simulink model "sim_tase_2025_pos_ctrl"  (R2020a)
settings: Solver=ode4  StartTime=0.0  StopTime=30.0  FixedStep=0.01  RelTol=1e-3
values from neighbouring files (symbols this model uses):
  alfa_theta_obs = 100    [init_tase_2025_pos_ctrl.m]
  Aps = -diag([5, 5, 5])    [init_tase_2025_pos_ctrl.m]
  delta_p_i_0 = zeros(3, NF)    [init_tase_2025_pos_ctrl.m]
  delta_v_i_0 = zeros(3, NF)    [init_tase_2025_pos_ctrl.m]
  dp_aa_t = 0.2 * ones(3, 5) + ( 1.0 - 0.2 ) * rand(3, 5)    [init_tase_2025_pos_ctrl.m]
  dp_ff_t = [ 0.4 * ones(1, 5) + ( 1.0 - 0.4 ) * rand(1, 5);                      0.4 * ones(1, 5) + ( 1.0 - 0.4 ) * rand(1, 5);                      0.2 * ones(1, 5) + ( 0.6 - 0.2 ) * rand(1, 5) ]    [init_tase_2025_pos_ctrl.m]
  dp_phi_t = ( - pi / 2 ) * ones(3, 5) + ( pi / 2 - ( - pi / 2 ) ) * rand(3, 5)    [init_tase_2025_pos_ctrl.m]
  etai_0 = zeros(3,5)    [init_tase_2025_pos_ctrl.m]
  k_rho_1 = 10    [init_tase_2025_pos_ctrl.m]
  k_rho_2 = 10    [init_tase_2025_pos_ctrl.m]
  kai_1_t = 0.02    [init_tase_2025_pos_ctrl.m]
  kai_3_t = 0.1    [init_tase_2025_pos_ctrl.m]
  kp = 20    [init_tase_2025_pos_ctrl.m]
  ksii_0 = zeros(3,5)    [init_tase_2025_pos_ctrl.m]
  kv = 20    [init_tase_2025_pos_ctrl.m]
  l1v = diag([20; 20; 20])    [init_tase_2025_pos_ctrl.m]
  l2v = diag([30; 30; 30])    [init_tase_2025_pos_ctrl.m]
  mass_i = zeros(1,NF)    [init_tase_2025_pos_ctrl.m]
  Mii = diag([1;0;0;0;1])    [init_tase_2025_pos_ctrl.m]
  Phi_inv = inv( Aps ) * ( exp( Aps * tTs ) - eye(3) )    [init_tase_2025_pos_ctrl.m]
  pos0 = zeros(3, 1)    [init_tase_2025_pos_ctrl.m]
  PZ0 = P0(3)    [init_tase_2025_pos_ctrl.m]
  PZ1 = 10    [init_tase_2025_pos_ctrl.m]
  Qci_init = repmat([1;0;0;0],1,NF)    [init_tase_2025_pos_ctrl.m]
  R0 = 4    [init_tase_2025_pos_ctrl.m]
  R1 = 8    [init_tase_2025_pos_ctrl.m]
  Rx2 = 10    [init_tase_2025_pos_ctrl.m]
  Ry2 = 6    [init_tase_2025_pos_ctrl.m]
  Rz2 = 4    [init_tase_2025_pos_ctrl.m]
  T0 = 0    [init_tase_2025_pos_ctrl.m]
  T1 = tseq1    (= 10)    [init_tase_2025_pos_ctrl.m]
  T12 = tseq1 + tseq12    (= 20)    [init_tase_2025_pos_ctrl.m]
  T2 = tseq1 + tseq12 + tseq2    (= 30)    [init_tase_2025_pos_ctrl.m]
  theta0 = ( 2 / 5 ) * pi    (= 1.25663706144)    [init_tase_2025_pos_ctrl.m]
  theta_1 = 0    [init_tase_2025_pos_ctrl.m]
  theta_2 = 1    [init_tase_2025_pos_ctrl.m]
  TTb = 2    [init_tase_2025_pos_ctrl.m]
  tTs = 0.1    [init_tase_2025_pos_ctrl.m]
  vel0 = zeros(3, 1)    [init_tase_2025_pos_ctrl.m]
  Wij = [0,0,1,0,0;              0,0,1,1,0;              1,0,0,0,1;              0,1,1,0,0;              0,0,1,0,0]    [init_tase_2025_pos_ctrl.m]
  wp = 10    [init_tase_2025_pos_ctrl.m]
  X1 = 8    [init_tase_2025_pos_ctrl.m]
  X2 = 2    [init_tase_2025_pos_ctrl.m]
  X3 = 3    [init_tase_2025_pos_ctrl.m]
  Y1 = 10    [init_tase_2025_pos_ctrl.m]
  Y2 = 2    [init_tase_2025_pos_ctrl.m]
  Y3 = 4    [init_tase_2025_pos_ctrl.m]
  Z1 = 4    [init_tase_2025_pos_ctrl.m]
  Z2 = -6    [init_tase_2025_pos_ctrl.m]
  Z3 = 2    [init_tase_2025_pos_ctrl.m]
undefined symbols (not defined in the file or in its folder): cal_frac_squ, p_gamma1_pos, p_gamma1_vel, p_gamma2_pos, p_gamma2_vel, p_gamma_diff_1, p_gamma_diff_2_2, q_gamma1_pos, q_gamma1_vel, q_gamma2_pos, q_gamma2_vel, q_gamma_diff_1, q_gamma_diff_2_2
(part 1 of 4)
settings Model: Creator=zzy  LastModifiedBy=Hershey.A
settings DataIOCC: ReturnWorkspaceOutputs=off
settings DebuggingCC: ArithmeticOperatorsInVariantConditions=warning
settings SFSimCC: SimUseLocalCustomCode=off  CustomCodeUndefinedFunction=UseInterfaceOnly
settings RTWCC: RTWUseLocalCustomCode=off

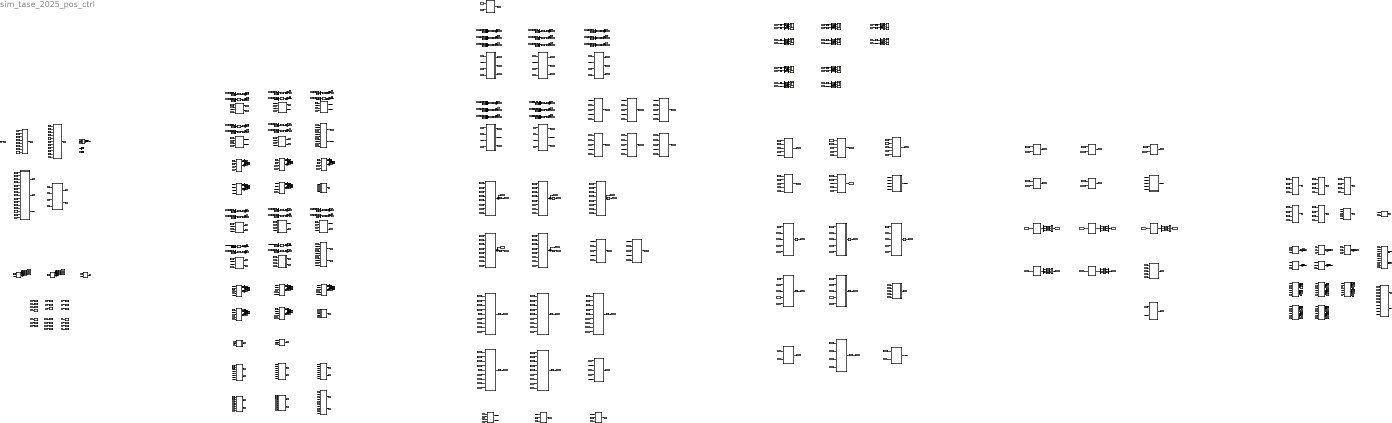
== system sim_tase_2025_pos_ctrl ==
  Add{,1..9} (10 alike) : Sum
  Clock : Clock
  Constant : Constant  Value=T1
  Constant{1,4,224,228,233,237,242} (7 alike) : Constant  Value=Mii
  Constant{6,8,10..11,13} (5 alike) : Constant  Value=kv
  Constant{28,34,40,46,100} (5 alike) : Constant
  Constant{59,65,74,79,88,90,92,96,101,106} (10 alike) : Constant  Value=TTb
  Constant{53..54,60,66,68,70,75,80,83,102} (10 alike) : Constant  Value=theta_1
  Constant{55,61,64,67,69,71,76,81,84,103} (10 alike) : Constant  Value=theta_2
  Constant{56..57,62,72,77,82,85..86,94,104} (10 alike) : Constant  Value=k_rho_1
  Constant{58,63,73,78,87,89,91,93,95,105} (10 alike) : Constant  Value=k_rho_2
  Constant{107,286,289,292,295} (5 alike) : Constant  Value=dp_phi_t
  Constant{108,287,290,293,296} (5 alike) : Constant  Value=dp_ff_t
  Constant109 : Constant  Value=R0
  Constant110 : Constant  Value=R1
  Constant111 : Constant  Value=T0
  Constant112 : Constant  Value=Rz2
  Constant113 : Constant  Value=Ry2
  Constant114 : Constant  Value=Rx2
  Constant115 : Constant  Value=X1
  Constant116 : Constant  Value=X2
  Constant117 : Constant  Value=Y1
  Constant118 : Constant  Value=Y2
  Constant119 : Constant  Value=T2
  Constant{3,7,9,12,14} (5 alike) : Constant  Value=kp
  Constant120 : Constant  Value=R0
  Constant121 : Constant  Value=R1
  Constant122 : Constant  Value=Rx2
  Constant123 : Constant  Value=Ry2
  Constant124 : Constant  Value=Rz2
  Constant125 : Constant  Value=T2
  Constant126 : Constant  Value=T1
  Constant127 : Constant  Value=PZ0
  Constant128 : Constant  Value=PZ1
  Constant{22..25,142} (5 alike) : Constant  Value=Phi_inv
  Constant{15..19,21} (6 alike) : Constant  Value=Aps
  Constant{182..183,189,199,202,205,209,212,219,252} (10 alike) : Constant  Value=l2v
  Constant{184..186,193..196,198,283..284} (10 alike) : Constant  Value=alfa_theta_obs
  Constant{187,190,197,200,203,206,210,213,230,263} (10 alike) : Constant  Value=l1v
  Constant188 : Constant  Value=delta_p_i_0(:,4)
  Constant191 : Constant  Value=mass_i
  Constant192 : Constant  Value=delta_p_i_0(:,5)
  Constant{2,5,223,227,232,236,240} (7 alike) : Constant  Value=Wij
  Constant20 : Constant  Value=tTs
  Constant201 : Constant  Value=delta_v_i_0(:,1)
  Constant204 : Constant  Value=delta_v_i_0(:,2)
  Constant207 : Constant  Value=delta_v_i_0(:,3)
  Constant208 : Constant  Value=delta_p_i_0(:,1)
  Constant211 : Constant  Value=delta_v_i_0(:,4)
  Constant214 : Constant  Value=delta_v_i_0(:,5)
  Constant{215,220,270,275,279} (5 alike) : Constant  Value=p_gamma1_pos
  Constant{216,267,271,276,280} (5 alike) : Constant  Value=q_gamma1_pos
  Constant{217,268,272,277,281} (5 alike) : Constant  Value=p_gamma2_pos
  Constant{218,269,273,278,282} (5 alike) : Constant  Value=q_gamma2_pos
  Constant221 : Constant  Value=Z1
  Constant222 : Constant  Value=Z2
  Constant225 : Constant  Value=theta0
  Constant226 : Constant  Value=Z3
  Constant229 : Constant  Value=Y3
  Constant231 : Constant  Value=kai_1_t
  Constant234 : Constant  Value=X3
  Constant235 : Constant  Value=kai_3_t
  Constant238 : Constant  Value=T1
  Constant239 : Constant  Value=T12
  Constant241 : Constant  Value=delta_p_i_0(:,2)
  Constant{245,249,254,258,262} (5 alike) : Constant  Value=p_gamma1_vel
  Constant{246,250,255,259,264} (5 alike) : Constant  Value=q_gamma1_vel
  Constant{247,251,256,260,265} (5 alike) : Constant  Value=p_gamma2_vel
  Constant{248,253,257,261,266} (5 alike) : Constant  Value=q_gamma2_vel
  Constant{26,29,35,41,47} (5 alike) : Constant  Value=p_gamma_diff_2_2
  Constant{27,30,36,42,48} (5 alike) : Constant  Value=q_gamma_diff_2_2
  Constant274 : Constant  Value=delta_p_i_0(:,3)
  Constant{285,288,291,294,297} (5 alike) : Constant  Value=dp_aa_t
  Constant{31,37,43,49,97} (5 alike) : Constant  Value=2
  Constant{32,38,44,50,98} (5 alike) : Constant  Value=p_gamma_diff_1
  Constant{33,39,45,52,99} (5 alike) : Constant  Value=q_gamma_diff_1
  Constant51 : Constant  Value=Qci_init
  Demux{,1..10,12,17..41,68..80,88,92..97} (57 alike) : Demux  Outputs=3
  Display{1..28,50..51,64..68,76..95} (55 alike) : Display
  Interpreted MATLAB Function{1..13,20..21,41..60} (35 alike) : MATLABFcn  MATLABFcn=cal_frac_squ(u(1:3),u(4),u(5))
  Memory1 : Memory  InitialCondition=etai_0
  Memory2 : Memory  InitialCondition=ksii_0
  Memory3 : Memory  InitialCondition=zeros(3,5)
  Mux{,1..4,7..12,19..27,109..118,120..129} (40 alike) : Mux  Inputs=3
  Mux{5..6,13..18,28..49,86..108,119,130..135} (60 alike) : Mux  Inputs=2
  Scope{4..13} (10 alike) : Scope  NumInputPorts=3
  Step : Step  Time=T1+0.01  SampleTime=0
  To Workspace : ToWorkspace  VariableName=eta_d_est_vec  SampleTime=-1
  To Workspace1 : ToWorkspace  VariableName=dp_hat_vec  SampleTime=-1
  To Workspace10 : ToWorkspace  VariableName=eta_track_err_vec  SampleTime=-1
  To Workspace11 : ToWorkspace  VariableName=sigma_bar_v_hat_vec  SampleTime=-1
  To Workspace12 : ToWorkspace  VariableName=sigma_bar_v_vec  SampleTime=-1
  To Workspace13 : ToWorkspace  VariableName=sigma_bar_v_tilt_vec  SampleTime=-1
  To Workspace14 : ToWorkspace  VariableName=ui  SampleTime=-1
  To Workspace17 : ToWorkspace  VariableName=ksi_est_err  SampleTime=-1
  To Workspace18 : ToWorkspace  VariableName=ksi_d_est_vec  SampleTime=-1
  To Workspace19 : ToWorkspace  VariableName=sigma_v_vec  SampleTime=-1
  To Workspace2 : ToWorkspace  VariableName=dp_vec  SampleTime=-1
  To Workspace20 : ToWorkspace  VariableName=vel_diff_hat_vec  SampleTime=-1
  To Workspace21 : ToWorkspace  VariableName=pos_diff_hat_vec  SampleTime=-1
  To Workspace22 : ToWorkspace  VariableName=eta_est_err  SampleTime=-1
  To Workspace3 : ToWorkspace  VariableName=u0  SampleTime=-1
  To Workspace4 : ToWorkspace  VariableName=eta0  SampleTime=-1
  To Workspace5 : ToWorkspace  VariableName=ksi0  SampleTime=-1
  To Workspace6 : ToWorkspace  VariableName=dp_tilt_vec  SampleTime=-1
  To Workspace7 : ToWorkspace  VariableName=eta_i_vec  SampleTime=-1
  To Workspace8 : ToWorkspace  VariableName=ksi_i_vec  SampleTime=-1
  To Workspace9 : ToWorkspace  VariableName=ksi_track_err_vec  SampleTime=-1
  Transfer Fcn{,1..14} (15 alike) : TransferFcn  Numerator=[wp]  Denominator=[1 wp]
  cal Rci from ui : MATLAB Function  TreatAsAtomicUnit=on
  cal Rei : MATLAB Function  TreatAsAtomicUnit=on
  cal Ri : MATLAB Function  TreatAsAtomicUnit=on
  cal abs 1 : MATLAB Function  TreatAsAtomicUnit=on
  cal abs 10 : MATLAB Function  TreatAsAtomicUnit=on
  cal abs 11 : MATLAB Function  TreatAsAtomicUnit=on
  cal abs 12 : MATLAB Function  TreatAsAtomicUnit=on
  cal abs 13 : MATLAB Function  TreatAsAtomicUnit=on
  cal abs 2 : MATLAB Function  TreatAsAtomicUnit=on
  cal abs 21 : MATLAB Function  TreatAsAtomicUnit=on
  cal abs 22 : MATLAB Function  TreatAsAtomicUnit=on
  cal abs 3 : MATLAB Function  TreatAsAtomicUnit=on
  cal abs 4 : MATLAB Function  TreatAsAtomicUnit=on
  cal abs 41 : MATLAB Function  TreatAsAtomicUnit=on
  cal abs 42 : MATLAB Function  TreatAsAtomicUnit=on
  cal abs 43 : MATLAB Function  TreatAsAtomicUnit=on
  cal abs 44 : MATLAB Function  TreatAsAtomicUnit=on
  cal abs 45 : MATLAB Function  TreatAsAtomicUnit=on
  cal abs 46 : MATLAB Function  TreatAsAtomicUnit=on
  cal abs 47 : MATLAB Function  TreatAsAtomicUnit=on
  cal abs 48 : MATLAB Function  TreatAsAtomicUnit=on
  cal abs 49 : MATLAB Function  TreatAsAtomicUnit=on
  cal abs 5 : MATLAB Function  TreatAsAtomicUnit=on
  cal abs 50 : MATLAB Function  TreatAsAtomicUnit=on
  cal abs 51 : MATLAB Function  TreatAsAtomicUnit=on
  cal abs 52 : MATLAB Function  TreatAsAtomicUnit=on
  cal abs 53 : MATLAB Function  TreatAsAtomicUnit=on
  cal abs 54 : MATLAB Function  TreatAsAtomicUnit=on
  cal abs 55 : MATLAB Function  TreatAsAtomicUnit=on
  cal abs 56 : MATLAB Function  TreatAsAtomicUnit=on
  cal abs 57 : MATLAB Function  TreatAsAtomicUnit=on
  cal abs 58 : MATLAB Function  TreatAsAtomicUnit=on
  cal abs 59 : MATLAB Function  TreatAsAtomicUnit=on
  cal abs 6 : MATLAB Function  TreatAsAtomicUnit=on
  cal abs 60 : MATLAB Function  TreatAsAtomicUnit=on
  cal abs 7 : MATLAB Function  TreatAsAtomicUnit=on
  cal abs 8 : MATLAB Function  TreatAsAtomicUnit=on
  cal abs 9 : MATLAB Function  TreatAsAtomicUnit=on
  cal control input ui : MATLAB Function  TreatAsAtomicUnit=on
  cal disturbance observation error dp_tilt : MATLAB Function  TreatAsAtomicUnit=on
  cal dp_hat agent 1 : MATLAB Function  TreatAsAtomicUnit=on
  cal dp_hat agent 2 : MATLAB Function  TreatAsAtomicUnit=on
  cal dp_hat agent 3 : MATLAB Function  TreatAsAtomicUnit=on
  cal dp_hat agent 4 : MATLAB Function  TreatAsAtomicUnit=on
  cal dp_hat agent 5 : MATLAB Function  TreatAsAtomicUnit=on
  cal formation tracking position errors : MATLAB Function  TreatAsAtomicUnit=on
  cal formation tracking velocity errors : MATLAB Function  TreatAsAtomicUnit=on
  cal high-order sliding mode differentiator position estimation error : MATLAB Function  TreatAsAtomicUnit=on
  cal lumped observation error agent 1 : MATLAB Function  TreatAsAtomicUnit=on
  cal lumped observation error agent 2 : MATLAB Function  TreatAsAtomicUnit=on
  cal lumped observation error agent 3 : MATLAB Function  TreatAsAtomicUnit=on
  cal lumped observation error agent 4 : MATLAB Function  TreatAsAtomicUnit=on
  cal lumped observation error agent 5 : MATLAB Function  TreatAsAtomicUnit=on
  cal mu_bTs_vec : MATLAB Function  TreatAsAtomicUnit=on
  cal pos_diff_hat agent 1 : MATLAB Function  TreatAsAtomicUnit=on
  cal pos_diff_hat agent 2 : MATLAB Function  TreatAsAtomicUnit=on
  cal pos_diff_hat agent 3 : MATLAB Function  TreatAsAtomicUnit=on
  cal pos_diff_hat agent 4 : MATLAB Function  TreatAsAtomicUnit=on
  cal pos_diff_hat agent 5 : MATLAB Function  TreatAsAtomicUnit=on
  cal position and velocity signal tracking errors : MATLAB Function  TreatAsAtomicUnit=on
  cal position estimate error : MATLAB Function  TreatAsAtomicUnit=on
  cal sample vl_tilt : MATLAB Function  TreatAsAtomicUnit=on
  cal sig_ksi_diff_tilt agent 1 : MATLAB Function  TreatAsAtomicUnit=on
  cal sig_ksi_diff_tilt agent 2 : MATLAB Function  TreatAsAtomicUnit=on
  cal sig_ksi_diff_tilt agent 3 : MATLAB Function  TreatAsAtomicUnit=on
  cal sig_ksi_diff_tilt agent 4 : MATLAB Function  TreatAsAtomicUnit=on
  cal sig_ksi_diff_tilt agent 5 : MATLAB Function  TreatAsAtomicUnit=on
  cal theta_eta_est_err_tilt agent 1 : MATLAB Function  TreatAsAtomicUnit=on
  cal theta_eta_est_err_tilt agent 2 : MATLAB Function  TreatAsAtomicUnit=on
  cal theta_eta_est_err_tilt agent 3 : MATLAB Function  TreatAsAtomicUnit=on
  cal theta_eta_est_err_tilt agent 4 : MATLAB Function  TreatAsAtomicUnit=on
  cal theta_eta_est_err_tilt agent 5 : MATLAB Function  TreatAsAtomicUnit=on
  cal theta_ksi_est_err_tilt agent 1 : MATLAB Function  TreatAsAtomicUnit=on
  cal theta_ksi_est_err_tilt agent 2 : MATLAB Function  TreatAsAtomicUnit=on
  cal theta_ksi_est_err_tilt agent 3 : MATLAB Function  TreatAsAtomicUnit=on
  cal theta_ksi_est_err_tilt agent 4 : MATLAB Function  TreatAsAtomicUnit=on
  cal theta_ksi_est_err_tilt agent 5 : MATLAB Function  TreatAsAtomicUnit=on
  cal ui0 agent 1 : MATLAB Function  TreatAsAtomicUnit=on
  cal ui0 agent 2 : MATLAB Function  TreatAsAtomicUnit=on
  cal ui0 agent 3 : MATLAB Function  TreatAsAtomicUnit=on
  cal ui0 agent 4 : MATLAB Function  TreatAsAtomicUnit=on
  cal ui0 agent 5 : MATLAB Function  TreatAsAtomicUnit=on
  cal vel_diff_hat agent 1 : MATLAB Function  TreatAsAtomicUnit=on
  cal vel_diff_hat agent 2 : MATLAB Function  TreatAsAtomicUnit=on
  cal vel_diff_hat agent 3 : MATLAB Function  TreatAsAtomicUnit=on
  cal vel_diff_hat agent 4 : MATLAB Function  TreatAsAtomicUnit=on
  cal vel_diff_hat agent 5 : MATLAB Function  TreatAsAtomicUnit=on
  cal velocity estimate error : MATLAB Function  TreatAsAtomicUnit=on
  cal vl_tilt prediction error : MATLAB Function  TreatAsAtomicUnit=on
  choose dp_hat agent 1 : MATLAB Function  TreatAsAtomicUnit=on
  choose dp_hat agent 2 : MATLAB Function  TreatAsAtomicUnit=on
  choose dp_hat agent 3 : MATLAB Function  TreatAsAtomicUnit=on
  choose dp_hat agent 4 : MATLAB Function  TreatAsAtomicUnit=on
  choose dp_hat agent 5 : MATLAB Function  TreatAsAtomicUnit=on
  choose eta_est_err_tilt 1 : MATLAB Function  TreatAsAtomicUnit=on
  choose eta_est_err_tilt 10 : MATLAB Function  TreatAsAtomicUnit=on
  choose eta_est_err_tilt 11 : MATLAB Function  TreatAsAtomicUnit=on
  choose eta_est_err_tilt 12 : MATLAB Function  TreatAsAtomicUnit=on
  choose eta_est_err_tilt 13 : MATLAB Function  TreatAsAtomicUnit=on
  choose eta_est_err_tilt 14 : MATLAB Function  TreatAsAtomicUnit=on
  choose eta_est_err_tilt 15 : MATLAB Function  TreatAsAtomicUnit=on
  choose eta_est_err_tilt 16 : MATLAB Function  TreatAsAtomicUnit=on
  choose eta_est_err_tilt 17 : MATLAB Function  TreatAsAtomicUnit=on
  choose eta_est_err_tilt 18 : MATLAB Function  TreatAsAtomicUnit=on
  choose eta_est_err_tilt 19 : MATLAB Function  TreatAsAtomicUnit=on
  choose eta_est_err_tilt 2 : MATLAB Function  TreatAsAtomicUnit=on
  choose eta_est_err_tilt 20 : MATLAB Function  TreatAsAtomicUnit=on
  choose eta_est_err_tilt 3 : MATLAB Function  TreatAsAtomicUnit=on
  choose eta_est_err_tilt 4 : MATLAB Function  TreatAsAtomicUnit=on
  choose eta_est_err_tilt 5 : MATLAB Function  TreatAsAtomicUnit=on
  choose eta_est_err_tilt 6 : MATLAB Function  TreatAsAtomicUnit=on
  choose eta_est_err_tilt 7 : MATLAB Function  TreatAsAtomicUnit=on
  choose eta_est_err_tilt 8 : MATLAB Function  TreatAsAtomicUnit=on
  choose eta_est_err_tilt 9 : MATLAB Function  TreatAsAtomicUnit=on
  choose eta_i agent 1 : MATLAB Function  TreatAsAtomicUnit=on
  choose eta_i agent 2 : MATLAB Function  TreatAsAtomicUnit=on
  choose eta_i agent 3 : MATLAB Function  TreatAsAtomicUnit=on
  choose eta_i agent 4 : MATLAB Function  TreatAsAtomicUnit=on
  choose eta_i agent 5 : MATLAB Function  TreatAsAtomicUnit=on
  choose ksi_diff_tilt : MATLAB Function  TreatAsAtomicUnit=on
  choose ksi_diff_tilt 1 : MATLAB Function  TreatAsAtomicUnit=on
  choose ksi_diff_tilt 10 : MATLAB Function  TreatAsAtomicUnit=on
  choose ksi_diff_tilt 2 : MATLAB Function  TreatAsAtomicUnit=on
  choose ksi_diff_tilt 3 : MATLAB Function  TreatAsAtomicUnit=on
  choose ksi_diff_tilt 4 : MATLAB Function  TreatAsAtomicUnit=on
  choose ksi_diff_tilt 5 : MATLAB Function  TreatAsAtomicUnit=on
  choose ksi_diff_tilt 6 : MATLAB Function  TreatAsAtomicUnit=on
  choose ksi_diff_tilt 7 : MATLAB Function  TreatAsAtomicUnit=on
  choose ksi_diff_tilt 8 : MATLAB Function  TreatAsAtomicUnit=on
  choose ksi_diff_tilt 9 : MATLAB Function  TreatAsAtomicUnit=on
  choose ksi_diff_tilt1 : MATLAB Function  TreatAsAtomicUnit=on
  choose ksi_diff_tilt2 : MATLAB Function  TreatAsAtomicUnit=on
  choose ksi_diff_tilt3 : MATLAB Function  TreatAsAtomicUnit=on
  choose ksi_diff_tilt4 : MATLAB Function  TreatAsAtomicUnit=on
  choose ksi_i agent 1 : MATLAB Function  TreatAsAtomicUnit=on
  choose ksi_i agent 2 : MATLAB Function  TreatAsAtomicUnit=on
  choose ksi_i agent 3 : MATLAB Function  TreatAsAtomicUnit=on
  choose ksi_i agent 4 : MATLAB Function  TreatAsAtomicUnit=on
  choose ksi_i agent 5 : MATLAB Function  TreatAsAtomicUnit=on
  choose pos_diff_hat agent 1 : MATLAB Function  TreatAsAtomicUnit=on
  choose pos_diff_hat agent 2 : MATLAB Function  TreatAsAtomicUnit=on
  choose pos_diff_hat agent 3 : MATLAB Function  TreatAsAtomicUnit=on
  choose pos_diff_hat agent 4 : MATLAB Function  TreatAsAtomicUnit=on
  choose pos_diff_hat agent 5 : MATLAB Function  TreatAsAtomicUnit=on
  choose vel_diff_hat agent 1 : MATLAB Function  TreatAsAtomicUnit=on
  choose vel_diff_hat agent 2 : MATLAB Function  TreatAsAtomicUnit=on
  choose vel_diff_hat agent 3 : MATLAB Function  TreatAsAtomicUnit=on
  choose vel_diff_hat agent 4 : MATLAB Function  TreatAsAtomicUnit=on
  choose vel_diff_hat agent 5 : MATLAB Function  TreatAsAtomicUnit=on
  combine d_vel_diff_hat : MATLAB Function  TreatAsAtomicUnit=on
  combine dp_hat : MATLAB Function  TreatAsAtomicUnit=on
  combine follower desire velocity estimaters : MATLAB Function  TreatAsAtomicUnit=on
  combine follower eta ksi : MATLAB Function  TreatAsAtomicUnit=on
  combine formation control input : MATLAB Function  TreatAsAtomicUnit=on
  combine ksi_diff_tilt_squ_1_2 : MATLAB Function  TreatAsAtomicUnit=on
  combine ksi_diff_tilt_squ_gamma_1 : MATLAB Function  TreatAsAtomicUnit=on
  combine ksi_diff_tilt_squ_gamma_2_2 : MATLAB Function  TreatAsAtomicUnit=on
  combine leader position estimaters : MATLAB Function  TreatAsAtomicUnit=on
  "combine lumped follower observation error " : MATLAB Function  TreatAsAtomicUnit=on
  combine lumped follower position observation error : MATLAB Function  TreatAsAtomicUnit=on
  combine lumped follower velocity observation error : MATLAB Function  TreatAsAtomicUnit=on
  combine pos_diff_hat : MATLAB Function  TreatAsAtomicUnit=on
  combine sig_ksi_diff_tilt_1_2 : MATLAB Function  TreatAsAtomicUnit=on
  combine sig_ksi_diff_tilt_gamma_1 : MATLAB Function  TreatAsAtomicUnit=on
  combine sig_ksi_diff_tilt_gamma_2_2 : MATLAB Function  TreatAsAtomicUnit=on
  combine translational disturbance : MATLAB Function  TreatAsAtomicUnit=on
  combine ui0 : MATLAB Function  TreatAsAtomicUnit=on
  combine ui1_vec : MATLAB Function  TreatAsAtomicUnit=on
  combine vel_diff_hat : MATLAB Function  TreatAsAtomicUnit=on
  combine vl_hat : MATLAB Function  TreatAsAtomicUnit=on
  depart Rc1 : MATLAB Function  TreatAsAtomicUnit=on
  depart Rc2 : MATLAB Function  TreatAsAtomicUnit=on
  depart Rc3 : MATLAB Function  TreatAsAtomicUnit=on
  depart Rc4 : MATLAB Function  TreatAsAtomicUnit=on
  depart Rc5 : MATLAB Function  TreatAsAtomicUnit=on
  depart Re1 : MATLAB Function  TreatAsAtomicUnit=on
  depart Re2 : MATLAB Function  TreatAsAtomicUnit=on
  depart Re3 : MATLAB Function  TreatAsAtomicUnit=on
  depart Re4 : MATLAB Function  TreatAsAtomicUnit=on
  depart Re5 : MATLAB Function  TreatAsAtomicUnit=on
  desire formation position and velocity : MATLAB Function  TreatAsAtomicUnit=on
  eta_0 : Scope  NumInputPorts=3
  eta_d_est_{1..5} (5 alike) : Scope  NumInputPorts=3
  eta_track_err_{1..5} (5 alike) : Scope  NumInputPorts=3
  fixed-time distributed follower desire position observer agent 1 : MATLAB Function  TreatAsAtomicUnit=on
  fixed-time distributed follower desire position observer agent 2 : MATLAB Function  TreatAsAtomicUnit=on
  fixed-time distributed follower desire position observer agent 3 : MATLAB Function  TreatAsAtomicUnit=on
  fixed-time distributed follower desire position observer agent 4 : MATLAB Function  TreatAsAtomicUnit=on
  fixed-time distributed follower desire position observer agent 5 : MATLAB Function  TreatAsAtomicUnit=on
  fixed-time distributed follower desire velocity observer agent 1 : MATLAB Function  TreatAsAtomicUnit=on
  fixed-time distributed follower desire velocity observer agent 2 : MATLAB Function  TreatAsAtomicUnit=on
  fixed-time distributed follower desire velocity observer agent 3 : MATLAB Function  TreatAsAtomicUnit=on
  fixed-time distributed follower desire velocity observer agent 4 : MATLAB Function  TreatAsAtomicUnit=on
  fixed-time distributed follower desire velocity observer agent 5 : MATLAB Function  TreatAsAtomicUnit=on
  follower etai Integrator agent 1 : Integrator  InitialCondition=etai_0(:,1)
  follower etai Integrator agent 2 : Integrator  InitialCondition=etai_0(:,2)
  follower etai Integrator agent 3 : Integrator  InitialCondition=etai_0(:,3)
  follower etai Integrator agent 4 : Integrator  InitialCondition=etai_0(:,4)
  follower etai Integrator agent 5 : Integrator  InitialCondition=etai_0(:,5)
  follower ksii Integrator agent 1 : Integrator  InitialCondition=ksii_0(:,1)
  follower ksii Integrator agent 2 : Integrator  InitialCondition=ksii_0(:,2)
  follower ksii Integrator agent 3 : Integrator  InitialCondition=ksii_0(:,3)
  follower ksii Integrator agent 4 : Integrator  InitialCondition=ksii_0(:,4)
  follower ksii Integrator agent 5 : Integrator  InitialCondition=ksii_0(:,5)
  follower tracking error agent 1 : MATLAB Function  TreatAsAtomicUnit=on
  follower tracking error agent 2 : MATLAB Function  TreatAsAtomicUnit=on
  follower tracking error agent 3 : MATLAB Function  TreatAsAtomicUnit=on
  follower tracking error agent 4 : MATLAB Function  TreatAsAtomicUnit=on
  follower tracking error agent 5 : MATLAB Function  TreatAsAtomicUnit=on
  generate translational disturbance agent 1 : MATLAB Function  TreatAsAtomicUnit=on
  generate translational disturbance agent 2 : MATLAB Function  TreatAsAtomicUnit=on
  generate translational disturbance agent 3 : MATLAB Function  TreatAsAtomicUnit=on
  generate translational disturbance agent 4 : MATLAB Function  TreatAsAtomicUnit=on
  generate translational disturbance agent 5 : MATLAB Function  TreatAsAtomicUnit=on
  ksi_0 : Scope  NumInputPorts=3
  ksi_d_est_{1..5} (5 alike) : Scope  NumInputPorts=3
  ksi_track_err_{1..5} (5 alike) : Scope  NumInputPorts=3
  leader control input : MATLAB Function  TreatAsAtomicUnit=on
  leader eta0 Integrator : Integrator  ExternalReset=rising  InitialConditionSource=external  InitialCondition=vel0
  leader ksi0 Integrator : Integrator  InitialCondition=pos0
  pos_diff_hat Integrator {1..5} (5 alike) : Integrator  InitialCondition=zeros(3,1)
  position observe Integrator {1..5} (5 alike) : Integrator  InitialCondition=zeros(3,1)
  process velocity : MATLAB Function  TreatAsAtomicUnit=on
  set desire formation configuration : MATLAB Function  TreatAsAtomicUnit=on
  trans to column1 : MATLAB Function  TreatAsAtomicUnit=on
  trans to column10 : MATLAB Function  TreatAsAtomicUnit=on
  trans to column11 : MATLAB Function  TreatAsAtomicUnit=on
  trans to column12 : MATLAB Function  TreatAsAtomicUnit=on
  trans to column13 : MATLAB Function  TreatAsAtomicUnit=on
  trans to column2 : MATLAB Function  TreatAsAtomicUnit=on
  trans to column20 : MATLAB Function  TreatAsAtomicUnit=on
  trans to column21 : MATLAB Function  TreatAsAtomicUnit=on
  trans to column3 : MATLAB Function  TreatAsAtomicUnit=on
  trans to column4 : MATLAB Function  TreatAsAtomicUnit=on
  trans to column41 : MATLAB Function  TreatAsAtomicUnit=on
  trans to column42 : MATLAB Function  TreatAsAtomicUnit=on
  trans to column43 : MATLAB Function  TreatAsAtomicUnit=on
  trans to column44 : MATLAB Function  TreatAsAtomicUnit=on
  trans to column45 : MATLAB Function  TreatAsAtomicUnit=on
  trans to column46 : MATLAB Function  TreatAsAtomicUnit=on
  trans to column47 : MATLAB Function  TreatAsAtomicUnit=on
  trans to column48 : MATLAB Function  TreatAsAtomicUnit=on
  trans to column49 : MATLAB Function  TreatAsAtomicUnit=on
  trans to column5 : MATLAB Function  TreatAsAtomicUnit=on
  trans to column50 : MATLAB Function  TreatAsAtomicUnit=on
  trans to column51 : MATLAB Function  TreatAsAtomicUnit=on
  trans to column52 : MATLAB Function  TreatAsAtomicUnit=on
  trans to column53 : MATLAB Function  TreatAsAtomicUnit=on
  trans to column54 : MATLAB Function  TreatAsAtomicUnit=on
  trans to column55 : MATLAB Function  TreatAsAtomicUnit=on
  trans to column56 : MATLAB Function  TreatAsAtomicUnit=on
  trans to column57 : MATLAB Function  TreatAsAtomicUnit=on
  trans to column58 : MATLAB Function  TreatAsAtomicUnit=on
  trans to column59 : MATLAB Function  TreatAsAtomicUnit=on
  trans to column6 : MATLAB Function  TreatAsAtomicUnit=on
  trans to column60 : MATLAB Function  TreatAsAtomicUnit=on
  trans to column7 : MATLAB Function  TreatAsAtomicUnit=on
  trans to column8 : MATLAB Function  TreatAsAtomicUnit=on
  trans to column9 : MATLAB Function  TreatAsAtomicUnit=on
  uav translational dynamics agent 1 : MATLAB Function  TreatAsAtomicUnit=on
  uav translational dynamics agent 2 : MATLAB Function  TreatAsAtomicUnit=on
  uav translational dynamics agent 3 : MATLAB Function  TreatAsAtomicUnit=on
  uav translational dynamics agent 4 : MATLAB Function  TreatAsAtomicUnit=on
  uav translational dynamics agent 5 : MATLAB Function  TreatAsAtomicUnit=on
  update vl_hat agent 1 : MATLAB Function  TreatAsAtomicUnit=on
  update vl_hat agent 2 : MATLAB Function  TreatAsAtomicUnit=on
  update vl_hat agent 3 : MATLAB Function  TreatAsAtomicUnit=on
  update vl_hat agent 4 : MATLAB Function  TreatAsAtomicUnit=on
  update vl_hat agent 5 : MATLAB Function  TreatAsAtomicUnit=on
  vel_diff_hat Integrator {1..5} (5 alike) : Integrator  InitialCondition=zeros(3,1)
  velocity observe Integrator {1..5} (5 alike) : Integrator  InitialCondition=zeros(3,1)
  vl_hat Integrator {1..5} (5 alike) : Integrator  InitialCondition=zeros(3,1)
  wires:
  follower etai Integrator agent 1/1 -> [eta_1], follower ksii Integrator agent 1/1
  follower etai Integrator agent 2/1 -> [eta_2], follower ksii Integrator agent 2/1
  follower etai Integrator agent 3/1 -> [eta_3], follower ksii Integrator agent 3/1
  follower etai Integrator agent 4/1 -> [eta_4], follower ksii Integrator agent 4/1
  follower etai Integrator agent 5/1 -> [eta_5], follower ksii Integrator agent 5/1
  follower ksii Integrator agent 1/1 -> [ksi_1]
  follower ksii Integrator agent 2/1 -> [ksi_2]
  follower ksii Integrator agent 3/1 -> [ksi_3]
  follower ksii Integrator agent 4/1 -> [ksi_4]
  follower ksii Integrator agent 5/1 -> [ksi_5]
  [eta_1] -> combine formation control input/1(eta_1)
  [eta_2] -> combine formation control input/2(eta_2)
  [eta_3] -> combine formation control input/3(eta_3)
  [eta_4] -> combine formation control input/4(eta_4)
  [eta_5] -> combine formation control input/5(eta_5)
  [ksi_1] -> combine formation control input/6(ksi_1)
  [ksi_2] -> combine formation control input/7(ksi_2)
  [ksi_3] -> combine formation control input/8(ksi_3)
  [ksi_4] -> combine formation control input/9(ksi_4)
  [ksi_5] -> combine formation control input/10(ksi_5)
  [ksi_i_vec] -> follower tracking error agent 1/3(ksi_i_vec)
  [eta_i_vec] -> follower tracking error agent 1/4(eta_i_vec)
  [ksi0] -> follower tracking error agent 1/5(ksi0)
  [eta0] -> follower tracking error agent 1/6(eta0)
  follower tracking error agent 1/2(eta_track_err_1) -> Display13/1, Demux24/1, [eta_track_err_1]
  follower tracking error agent 1/1(ksi_track_err_1) -> Display12/1, Demux23/1, [ksi_track_err_1]
  [eta0] -> follower tracking error agent 2/6(eta0)
  [ksi0] -> follower tracking error agent 2/5(ksi0)
  [eta_i_vec] -> follower tracking error agent 2/4(eta_i_vec)
  follower tracking error agent 2/2(eta_track_err_2) -> Display15/1, Demux26/1, [eta_track_err_2]
  [ksi_i_vec] -> follower tracking error agent 2/3(ksi_i_vec)
  follower tracking error agent 2/1(ksi_track_err_2) -> Display14/1, Demux25/1, [ksi_track_err_2]
  follower tracking error agent 3/2(eta_track_err_3) -> Display17/1, Demux28/1, [eta_track_err_3]
  follower tracking error agent 3/1(ksi_track_err_3) -> Display16/1, Demux27/1, [ksi_track_err_3]
  [eta0] -> follower tracking error agent 3/6(eta0)
  [eta_i_vec] -> follower tracking error agent 3/4(eta_i_vec)
  [ksi_i_vec] -> follower tracking error agent 3/3(ksi_i_vec)
  [ksi0] -> follower tracking error agent 3/5(ksi0)
  [ksi_i_vec] -> follower tracking error agent 4/3(ksi_i_vec)
  [ksi0] -> follower tracking error agent 4/5(ksi0)
  [eta_i_vec] -> follower tracking error agent 4/4(eta_i_vec)
  [eta0] -> follower tracking error agent 4/6(eta0)
  follower tracking error agent 4/2(eta_track_err_4) -> Display19/1, Demux30/1, [eta_track_err_4]
  follower tracking error agent 4/1(ksi_track_err_4) -> Display18/1, Demux29/1, [ksi_track_err_4]
  follower tracking error agent 5/1(ksi_track_err_5) -> Display20/1, Demux31/1, [ksi_track_err_5]
  [ksi_i_vec] -> follower tracking error agent 5/3(ksi_i_vec)
  [eta0] -> follower tracking error agent 5/6(eta0)
  [ksi0] -> follower tracking error agent 5/5(ksi0)
  [eta_i_vec] -> follower tracking error agent 5/4(eta_i_vec)
  follower tracking error agent 5/2(eta_track_err_5) -> Display21/1, Demux32/1, [eta_track_err_5]
  [ksi_track_err_1] -> combine follower eta ksi/1(ksi_track_err_1)
  [ksi_track_err_2] -> combine follower eta ksi/2(ksi_track_err_2)
  [ksi_track_err_3] -> combine follower eta ksi/3(ksi_track_err_3)
  [ksi_track_err_4] -> combine follower eta ksi/4(ksi_track_err_4)
  [ksi_track_err_5] -> combine follower eta ksi/5(ksi_track_err_5)
  [eta_track_err_1] -> combine follower eta ksi/6(eta_track_err_1)
  [eta_track_err_2] -> combine follower eta ksi/7(eta_track_err_2)
  [eta_track_err_3] -> combine follower eta ksi/8(eta_track_err_3)
  [eta_track_err_4] -> combine follower eta ksi/9(eta_track_err_4)
  [eta_track_err_5] -> combine follower eta ksi/10(eta_track_err_5)
  combine follower eta ksi/1(ksi_track_err_vec) -> [ksi_track_err_vec]
  combine follower eta ksi/2(eta_track_err_vec) -> [eta_track_err_vec]
  Demux23/2 -> ksi_track_err_1/2
  Demux23/1 -> ksi_track_err_1/1
  Demux23/3 -> ksi_track_err_1/3
  Demux24/2 -> eta_track_err_1/2
  Demux24/1 -> eta_track_err_1/1
  Demux24/3 -> eta_track_err_1/3
  Demux25/2 -> ksi_track_err_2/2
  Demux25/1 -> ksi_track_err_2/1
  Demux25/3 -> ksi_track_err_2/3
  Demux26/1 -> eta_track_err_2/1
  Demux26/3 -> eta_track_err_2/3
  Demux26/2 -> eta_track_err_2/2
  Demux27/1 -> ksi_track_err_3/1
  Demux27/3 -> ksi_track_err_3/3
  Demux27/2 -> ksi_track_err_3/2
  Demux28/3 -> eta_track_err_3/3
  Demux28/2 -> eta_track_err_3/2
  Demux28/1 -> eta_track_err_3/1
  Demux29/3 -> ksi_track_err_4/3
  Demux29/2 -> ksi_track_err_4/2
  Demux29/1 -> ksi_track_err_4/1
  Demux30/3 -> eta_track_err_4/3
  Demux30/2 -> eta_track_err_4/2
  Demux30/1 -> eta_track_err_4/1
  Demux31/3 -> ksi_track_err_5/3
  Demux31/2 -> ksi_track_err_5/2
  Demux31/1 -> ksi_track_err_5/1
  Demux32/3 -> eta_track_err_5/3
  Demux32/2 -> eta_track_err_5/2
  Demux32/1 -> eta_track_err_5/1
  combine formation control input/1(eta_i_vec) -> Memory1/1
  Memory1/1 -> [eta_i_vec]
  combine formation control input/2(ksi_i_vec) -> Memory2/1
  Memory2/1 -> [ksi_i_vec]
  [ui] -> uav translational dynamics agent 1/2(ui)
  [Ri] -> uav translational dynamics agent 1/1(Ri)
  uav translational dynamics agent 1/1(dvi) -> follower etai Integrator agent 1/1
  uav translational dynamics agent 2/1(dvi) -> follower etai Integrator agent 2/1
  [ui] -> uav translational dynamics agent 2/2(ui)
  [Ri] -> uav translational dynamics agent 2/1(Ri)
  [ui] -> uav translational dynamics agent 3/2(ui)
  [Ri] -> uav translational dynamics agent 3/1(Ri)
  uav translational dynamics agent 3/1(dvi) -> follower etai Integrator agent 3/1
  [ui] -> uav translational dynamics agent 4/2(ui)
  [Ri] -> uav translational dynamics agent 4/1(Ri)
  uav translational dynamics agent 4/1(dvi) -> follower etai Integrator agent 4/1
  [ui] -> uav translational dynamics agent 5/2(ui)
  [Ri] -> uav translational dynamics agent 5/1(Ri)
  uav translational dynamics agent 5/1(dvi) -> follower etai Integrator agent 5/1
  [ui] -> cal Rci from ui/2(ui)
  Constant191/1 -> cal Rci from ui/1(mi)
  cal Rei/1(Rei) -> depart Re5/1(x), depart Re4/1(x), depart Re3/1(x), depart Re2/1(x), depart Re1/1(x), [Rei]
  depart Re2/1(y) -> Display65/1
  depart Re3/1(y) -> Display66/1
  depart Re1/1(y) -> Display64/1
  depart Re4/1(y) -> Display67/1
  Constant51/1 -> cal Rei/1(Qei)
  depart Re5/1(y) -> Display68/1
  [Rei] -> cal Ri/1(Rei)
  [Rci] -> cal Ri/2(Rci)
  cal Ri/1(Ri) -> [Ri]
  depart Rc5/1(y) -> Display25/1
  depart Rc2/1(y) -> Display22/1
  depart Rc3/1(y) -> Display23/1
  depart Rc4/1(y) -> Display24/1
  depart Rc1/1(y) -> Display6/1
  cal Rci from ui/1(Rci) -> [Rci], depart Rc5/1(x), depart Rc4/1(x), depart Rc3/1(x), depart Rc2/1(x), depart Rc1/1(x)
  [dp_vec] -> uav translational dynamics agent 1/3(dpi_vec)
  [dp_vec] -> uav translational dynamics agent 2/3(dpi_vec)
  [dp_vec] -> uav translational dynamics agent 3/3(dpi_vec)
  [dp_vec] -> uav translational dynamics agent 4/3(dpi_vec)
  [dp_vec] -> uav translational dynamics agent 5/3(dpi_vec)
  cal ui0 agent 1/1(ui0_1) -> [ui0_1]
  [ui0_5] -> combine ui0/5(ui0_5)
  [ui0_2] -> combine ui0/2(ui0_2)
  [ui0_1] -> combine ui0/1(ui0_1)
  [ui0_4] -> combine ui0/4(ui0_4)
  [ui0_3] -> combine ui0/3(ui0_3)
  [dp_vec] -> cal disturbance observation error dp_tilt/1(dp_vec)
  [dp_hat_vec] -> cal disturbance observation error dp_tilt/2(dp_hat_vec)
  cal disturbance observation error dp_tilt/1(dp_tilt_vec) -> [dp_tilt_vec]
  [eta_i_vec] -> cal position and velocity signal tracking errors/3(eta_i_vec)
  [ksi_i_vec] -> cal position and velocity signal tracking errors/1(ksi_i_vec)
  [ksi_d_est_vec] -> cal position and velocity signal tracking errors/2(ksi_d_est_vec)
  [eta_d_est_vec] -> cal position and velocity signal tracking errors/4(eta_d_est_vec)
  Constant4/1 -> cal formation tracking position errors/1(wi0)
  Constant5/1 -> cal formation tracking position errors/2(wij)
  cal position and velocity signal tracking errors/1(err_ksi_vec) -> [err_ksi_vec]
  [err_ksi_vec] -> cal formation tracking position errors/3(err_ksi_vec)
  cal formation tracking position errors/1(err_ksi_form_vec) -> [err_ksi_form_vec]
  cal position and velocity signal tracking errors/2(err_eta_vec) -> [err_eta_vec]
  cal formation tracking velocity errors/1(err_eta_form_vec) -> [err_eta_form_vec]
  [err_eta_vec] -> cal formation tracking velocity errors/3(err_eta_vec)
  Constant2/1 -> cal formation tracking velocity errors/2(wij)
  Constant1/1 -> cal formation tracking velocity errors/1(wi0)
  combine ui0/1(ui0) -> [ui0]
  Constant3/1 -> cal ui0 agent 1/1(kp)
  Constant6/1 -> cal ui0 agent 1/2(kv)
  [u0] -> cal ui0 agent 1/3(u0)
  [err_ksi_form_vec] -> cal ui0 agent 1/4(err_ksi_form_vec)
  [err_eta_form_vec] -> cal ui0 agent 1/5(err_eta_form_vec)
  Constant8/1 -> cal ui0 agent 2/2(kv)
  [err_eta_form_vec] -> cal ui0 agent 2/5(err_eta_form_vec)
  Constant7/1 -> cal ui0 agent 2/1(kp)
  [err_ksi_form_vec] -> cal ui0 agent 2/4(err_ksi_form_vec)
  cal ui0 agent 2/1(ui0_2) -> [ui0_2]
  [u0] -> cal ui0 agent 2/3(u0)
  cal ui0 agent 3/1(ui0_3) -> [ui0_3]
  [u0] -> cal ui0 agent 3/3(u0)
  [err_ksi_form_vec] -> cal ui0 agent 3/4(err_ksi_form_vec)
  Constant9/1 -> cal ui0 agent 3/1(kp)
  [err_eta_form_vec] -> cal ui0 agent 3/5(err_eta_form_vec)
  Constant10/1 -> cal ui0 agent 3/2(kv)
  Constant12/1 -> cal ui0 agent 4/1(kp)
  Constant11/1 -> cal ui0 agent 4/2(kv)
  [u0] -> cal ui0 agent 4/3(u0)
  cal ui0 agent 4/1(ui0_4) -> [ui0_4]
  [err_ksi_form_vec] -> cal ui0 agent 4/4(err_ksi_form_vec)
  [err_eta_form_vec] -> cal ui0 agent 4/5(err_eta_form_vec)
  [u0] -> cal ui0 agent 5/3(u0)
  cal ui0 agent 5/1(ui0_5) -> [ui0_5]
  Constant13/1 -> cal ui0 agent 5/2(kv)
  [err_ksi_form_vec] -> cal ui0 agent 5/4(err_ksi_form_vec)
  [err_eta_form_vec] -> cal ui0 agent 5/5(err_eta_form_vec)
  Constant14/1 -> cal ui0 agent 5/1(kp)
  Constant15/1 -> update vl_hat agent 1/1(Aps)
  [ui0] -> update vl_hat agent 1/2(ui0)
  [ui1] -> update vl_hat agent 1/3(ui1)
  [dp_hat_vec] -> update vl_hat agent 1/4(dp_hat_vec)
  [vl_tilt_vec] -> update vl_hat agent 1/5(vli_tilt_vec)
  update vl_hat agent 1/1(d_vl_hat_1) -> vl_hat Integrator 1/1
  vl_hat Integrator 1/1 -> [vl_hat_1]
  vl_hat Integrator 2/1 -> [vl_hat_2]
  Constant16/1 -> update vl_hat agent 2/1(Aps)
  [ui1] -> update vl_hat agent 2/3(ui1)
  [ui0] -> update vl_hat agent 2/2(ui0)
  [vl_tilt_vec] -> update vl_hat agent 2/5(vli_tilt_vec)
  update vl_hat agent 2/1(d_vl_hat_2) -> vl_hat Integrator 2/1
  [dp_hat_vec] -> update vl_hat agent 2/4(dp_hat_vec)
  update vl_hat agent 3/1(d_vl_hat_3) -> vl_hat Integrator 3/1
  [dp_hat_vec] -> update vl_hat agent 3/4(dp_hat_vec)
  vl_hat Integrator 3/1 -> [vl_hat_3]
  [vl_tilt_vec] -> update vl_hat agent 3/5(vli_tilt_vec)
  [ui0] -> update vl_hat agent 3/2(ui0)
  [ui1] -> update vl_hat agent 3/3(ui1)
  Constant17/1 -> update vl_hat agent 3/1(Aps)
  Constant18/1 -> update vl_hat agent 4/1(Aps)
  [ui1] -> update vl_hat agent 4/3(ui1)
  [vl_tilt_vec] -> update vl_hat agent 4/5(vli_tilt_vec)
  update vl_hat agent 4/1(d_vl_hat_4) -> vl_hat Integrator 4/1
  [ui0] -> update vl_hat agent 4/2(ui0)
  [dp_hat_vec] -> update vl_hat agent 4/4(dp_hat_vec)
  vl_hat Integrator 4/1 -> [vl_hat_4]
  [dp_hat_vec] -> update vl_hat agent 5/4(dp_hat_vec)
  vl_hat Integrator 5/1 -> [vl_hat_5]
  [ui1] -> update vl_hat agent 5/3(ui1)
  [vl_tilt_vec] -> update vl_hat agent 5/5(vli_tilt_vec)
  update vl_hat agent 5/1(d_vl_hat_5) -> vl_hat Integrator 5/1
  [ui0] -> update vl_hat agent 5/2(ui0)
  Constant19/1 -> update vl_hat agent 5/1(Aps)
  [vl_hat_3] -> combine vl_hat/3(vl_hat_3)
  [vl_hat_2] -> combine vl_hat/2(vl_hat_2)
  combine vl_hat/1(vl_hat_vec) -> [vl_hat_vec]
  [vl_hat_4] -> combine vl_hat/4(vl_hat_4)
  [vl_hat_5] -> combine vl_hat/5(vl_hat_5)
  [vl_hat_1] -> combine vl_hat/1(vl_hat_1)
  [eta_i_vec] -> cal vl_tilt prediction error/1(eta_i_vec)
  [vl_hat_vec] -> cal vl_tilt prediction error/2(vl_hat_vec)
  cal vl_tilt prediction error/1(vl_tilt_vec) -> [vl_tilt_vec]
  [tsim] -> cal sample vl_tilt/2(tsim)
  Constant20/1 -> cal sample vl_tilt/1(tTs)
  [vl_tilt_vec] -> cal sample vl_tilt/3(vl_tilt_vec)
  [vl_tilt_bTs_vec] -> cal sample vl_tilt/4("vl_tilt_bTs_vec ")
  cal sample vl_tilt/1(vl_tilt_bTs_vec) -> Memory3/1
  Memory3/1 -> [vl_tilt_bTs_vec]
  [vl_tilt_bTs_vec] -> cal mu_bTs_vec/2(vl_tilt_bTs_vec)
  Constant21/1 -> cal mu_bTs_vec/1(Aps)
  cal mu_bTs_vec/1(mu_bTs_vec) -> [mu_bTs_vec]
  [dp_hat_4] -> combine dp_hat/4(dp_hat_4)
  [dp_hat_2] -> combine dp_hat/2(dp_hat_2)
  [dp_hat_1] -> combine dp_hat/1(dp_hat_1)
  combine dp_hat/1(dp_hat_vec) -> [dp_hat_vec]
  cal dp_hat agent 1/1(dp_hat_1) -> [dp_hat_1]
  [dp_hat_3] -> combine dp_hat/3(dp_hat_3)
  [dp_hat_5] -> combine dp_hat/5(dp_hat_5)
  Constant142/1 -> cal dp_hat agent 1/1(Phi_inv)
  [mu_bTs_vec] -> cal dp_hat agent 1/2(mu_bTs_vec)
  [mu_bTs_vec] -> cal dp_hat agent 2/2(mu_bTs_vec)
  Constant22/1 -> cal dp_hat agent 2/1(Phi_inv)
  cal dp_hat agent 2/1(dp_hat_2) -> [dp_hat_2]
  cal dp_hat agent 3/1(dp_hat_3) -> [dp_hat_3]
  Constant23/1 -> cal dp_hat agent 3/1(Phi_inv)
  [mu_bTs_vec] -> cal dp_hat agent 3/2(mu_bTs_vec)
  Constant24/1 -> cal dp_hat agent 4/1(Phi_inv)
  [mu_bTs_vec] -> cal dp_hat agent 4/2(mu_bTs_vec)
  cal dp_hat agent 4/1(dp_hat_4) -> [dp_hat_4]
  Constant25/1 -> cal dp_hat agent 5/1(Phi_inv)
  cal dp_hat agent 5/1(dp_hat_5) -> [dp_hat_5]
  [mu_bTs_vec] -> cal dp_hat agent 5/2(mu_bTs_vec)
  [mu_bTs_vec] -> choose dp_hat agent 1/1(x)
  [mu_bTs_vec] -> choose dp_hat agent 2/1(x)
  [mu_bTs_vec] -> choose dp_hat agent 3/1(x)
  [mu_bTs_vec] -> choose dp_hat agent 4/1(x)
  [mu_bTs_vec] -> choose dp_hat agent 5/1(x)
  [ui1_5] -> combine ui1_vec/5(ui1_5)
  [ui1_3] -> combine ui1_vec/3(ui1_3)
  [ui1_1] -> combine ui1_vec/1(ui1_1)
  combine ui1_vec/1(ui1) -> [ui1]
  [ui1_2] -> combine ui1_vec/2(ui1_2)
  [ui1_4] -> combine ui1_vec/4(ui1_4)
  [ui0] -> cal control input ui/1(ui0)
  [ui1] -> cal control input ui/2(ui1)
  cal control input ui/1(ui) -> [ui]
  choose dp_hat agent 1/1(y) -> Demux/1
  Demux/1 -> Transfer Fcn/1
  Transfer Fcn/1 -> Mux/1
  Transfer Fcn5/1 -> Mux/2
  Mux/1 -> [ui1_1]
  Demux/2 -> Transfer Fcn5/1
  Demux/3 -> Transfer Fcn6/1
  Transfer Fcn6/1 -> Mux/3
  Transfer Fcn8/1 -> Mux1/3
  Mux1/1 -> [ui1_2]
  Transfer Fcn1/1 -> Mux1/1
  Transfer Fcn7/1 -> Mux1/2
  Demux2/2 -> Transfer Fcn7/1
  Demux2/1 -> Transfer Fcn1/1
  Demux2/3 -> Transfer Fcn8/1
  choose dp_hat agent 2/1(y) -> Demux2/1
  Transfer Fcn4/1 -> Mux2/3
  Mux2/1 -> [ui1_3]
  Transfer Fcn2/1 -> Mux2/1
  Transfer Fcn3/1 -> Mux2/2
  Demux3/2 -> Transfer Fcn3/1
  Demux3/1 -> Transfer Fcn2/1
  Demux3/3 -> Transfer Fcn4/1
  choose dp_hat agent 3/1(y) -> Demux3/1
  Transfer Fcn11/1 -> Mux3/3
  Mux3/1 -> [ui1_4]
  Transfer Fcn9/1 -> Mux3/1
  Transfer Fcn10/1 -> Mux3/2
  Demux4/2 -> Transfer Fcn10/1
  Demux4/1 -> Transfer Fcn9/1
  Demux4/3 -> Transfer Fcn11/1
  choose dp_hat agent 4/1(y) -> Demux4/1
  Transfer Fcn14/1 -> Mux4/3
  Mux4/1 -> [ui1_5]
  Transfer Fcn12/1 -> Mux4/1
  Transfer Fcn13/1 -> Mux4/2
  Demux5/2 -> Transfer Fcn13/1
  Demux5/1 -> Transfer Fcn12/1
  Demux5/3 -> Transfer Fcn14/1
  choose dp_hat agent 5/1(y) -> Demux5/1
  cal sig_ksi_diff_tilt agent 5/2(sig_ksi_diff_tilt_gamma_1_node_5) -> [sig_ksi_diff_tilt_gamma_1_node_5]
  [ksi_diff_tilt_squ_gamma_1_node_4] -> combine ksi_diff_tilt_squ_gamma_1/4(ksi_diff_tilt_squ_gamma_1_node_4)
  trans to column9/1(y) -> [ksi_diff_tilt_squ_gamma_1_node_4], Display10/1
  cal sig_ksi_diff_tilt agent 1/2(sig_ksi_diff_tilt_gamma_1_node_1) -> [sig_ksi_diff_tilt_gamma_1_node_1]
  [ksi_diff_tilt_vec] -> choose ksi_diff_tilt 1/1(x)
  Constant100/1 -> Mux22/2
  [ksi_i_vec] -> cal high-order sliding mode differentiator position estimation error/1(ksi_i_vec)
  trans to column2/1(y) -> [ksi_diff_tilt_squ_gamma_2_2_node_2], Display2/1
  choose ksi_diff_tilt 2/1(y) -> cal abs 1/1(x)
  Mux21/1 -> Interpreted MATLAB Function20/1
  choose ksi_diff_tilt 10/1(y) -> cal abs 12/1(x)
  [ksi_diff_tilt_vec] -> choose ksi_diff_tilt/1(x)
  [ksi_diff_tilt_squ_1_2_node_1] -> combine ksi_diff_tilt_squ_1_2/1(ksi_diff_tilt_squ_1_2_node_1)
  Constant44/1 -> Mux8/2
  choose ksi_diff_tilt1/1(y) -> cal abs 3/1(x)
  [sig_ksi_diff_tilt_1_2_node_2] -> combine sig_ksi_diff_tilt_1_2/2(sig_ksi_diff_tilt_1_2_node_2)
  cal abs 22/1(y) -> Mux21/1
  [sig_ksi_diff_tilt_gamma_2_2_node_1] -> combine sig_ksi_diff_tilt_gamma_2_2/1(sig_ksi_diff_tilt_gamma_2_2_node_1)
  cal abs 3/1(y) -> Mux25/1
  trans to column1/1(y) -> [ksi_diff_tilt_squ_gamma_2_2_node_1], Display1/1
  choose ksi_diff_tilt 9/1(y) -> cal abs 11/1(x)
  Mux9/1 -> Interpreted MATLAB Function11/1
  Constant52/1 -> Mux20/3
  choose ksi_diff_tilt 8/1(y) -> cal abs 8/1(x)
  trans to column12/1(y) -> [ksi_diff_tilt_squ_gamma_2_2_node_5], Display28/1
  choose ksi_diff_tilt 3/1(y) -> cal abs 4/1(x)
  [ksi_diff_tilt_vec] -> choose ksi_diff_tilt 8/1(x)
  [ksi_diff_tilt_squ_1_2_node_5] -> combine ksi_diff_tilt_squ_1_2/5(ksi_diff_tilt_squ_1_2_node_5)
  Constant48/1 -> Mux19/3
  cal sig_ksi_diff_tilt agent 1/3(sig_ksi_diff_tilt_gamma_2_2_node_1) -> [sig_ksi_diff_tilt_gamma_2_2_node_1]
  Interpreted MATLAB Function1/1 -> trans to column1/1(x)
  cal abs 13/1(y) -> Mux9/1
  choose ksi_diff_tilt 1/1(y) -> cal abs 22/1(x)
  trans to column3/1(y) -> [ksi_diff_tilt_squ_gamma_1_node_2], Display3/1
  [ksi_diff_tilt_squ_gamma_1_node_5] -> combine ksi_diff_tilt_squ_gamma_1/5(ksi_diff_tilt_squ_gamma_1_node_5)
  Mux22/1 -> Interpreted MATLAB Function21/1
  Constant99/1 -> Mux21/3
  combine ksi_diff_tilt_squ_gamma_1/1(ksi_diff_tilt_squ_gamma_1_vec) -> [ksi_diff_tilt_squ_gamma_1_vec]
  [ksi_diff_tilt_squ_gamma_2_2_node_5] -> combine ksi_diff_tilt_squ_gamma_2_2/5(ksi_diff_tilt_squ_gamma_2_2_node_5)
  [ksi_diff_tilt_squ_gamma_1_node_2] -> combine ksi_diff_tilt_squ_gamma_1/2(ksi_diff_tilt_squ_gamma_1_node_2)
  [ksi_diff_tilt_vec] -> cal sig_ksi_diff_tilt agent 2/1(ksi_diff_tilt_vec)
  choose ksi_diff_tilt 7/1(y) -> cal abs 10/1(x)
  [ksi_diff_tilt_squ_gamma_1_node_1] -> combine ksi_diff_tilt_squ_gamma_1/1(ksi_diff_tilt_squ_gamma_1_node_1)
  cal sig_ksi_diff_tilt agent 4/2(sig_ksi_diff_tilt_gamma_1_node_4) -> [sig_ksi_diff_tilt_gamma_1_node_4]
  [ksi_diff_tilt_squ_1_2_node_4] -> combine ksi_diff_tilt_squ_1_2/4(ksi_diff_tilt_squ_1_2_node_4)
  [ksi_diff_tilt_squ_1_2_vec] -> cal sig_ksi_diff_tilt agent 1/2(ksi_diff_tilt_squ_1_2_vec)
  [ksi_diff_tilt_squ_1_2_node_3] -> combine ksi_diff_tilt_squ_1_2/3(ksi_diff_tilt_squ_1_2_node_3)
  Constant31/1 -> Mux25/3
  trans to column8/1(y) -> [ksi_diff_tilt_squ_gamma_2_2_node_4], Display9/1
  [sig_ksi_diff_tilt_gamma_2_2_node_4] -> combine sig_ksi_diff_tilt_gamma_2_2/4(sig_ksi_diff_tilt_gamma_2_2_node_4)
  [sig_ksi_diff_tilt_gamma_1_node_3] -> combine sig_ksi_diff_tilt_gamma_1/3(sig_ksi_diff_tilt_gamma_1_node_3)
  [ksi_diff_tilt_vec] -> choose ksi_diff_tilt 7/1(x)
  [ksi_diff_tilt_squ_gamma_2_2_node_2] -> combine ksi_diff_tilt_squ_gamma_2_2/2(ksi_diff_tilt_squ_gamma_2_2_node_2)
  combine sig_ksi_diff_tilt_1_2/1(sig_ksi_diff_tilt_1_2_vec) -> [sig_ksi_diff_tilt_1_2_vec]
  [ksi_diff_tilt_squ_1_2_node_2] -> combine ksi_diff_tilt_squ_1_2/2(ksi_diff_tilt_squ_1_2_node_2)
  [sig_ksi_diff_tilt_1_2_node_4] -> combine sig_ksi_diff_tilt_1_2/4(sig_ksi_diff_tilt_1_2_node_4)
  trans to column4/1(y) -> [ksi_diff_tilt_squ_1_2_node_2], Display4/1
  combine ksi_diff_tilt_squ_1_2/1(ksi_diff_tilt_squ_1_2_vec) -> [ksi_diff_tilt_squ_1_2_vec]
  Mux26/1 -> Interpreted MATLAB Function2/1
  [ksi_diff_tilt_squ_gamma_2_2_vec] -> cal sig_ksi_diff_tilt agent 1/4(ksi_diff_tilt_squ_gamma_2_2_vec)
  [ksi_diff_tilt_squ_gamma_1_vec] -> cal sig_ksi_diff_tilt agent 5/3(ksi_diff_tilt_squ_gamma_1_vec)
  Interpreted MATLAB Function3/1 -> trans to column3/1(x)
  [ksi_diff_tilt_squ_gamma_2_2_node_1] -> combine ksi_diff_tilt_squ_gamma_2_2/1(ksi_diff_tilt_squ_gamma_2_2_node_1)
  [ksi_diff_tilt_squ_gamma_1_vec] -> cal sig_ksi_diff_tilt agent 2/3(ksi_diff_tilt_squ_gamma_1_vec)
  [sig_ksi_diff_tilt_1_2_node_3] -> combine sig_ksi_diff_tilt_1_2/3(sig_ksi_diff_tilt_1_2_node_3)
  cal sig_ksi_diff_tilt agent 2/3(sig_ksi_diff_tilt_gamma_2_2_node_2) -> [sig_ksi_diff_tilt_gamma_2_2_node_2]
  [ksi_diff_tilt_squ_gamma_2_2_vec] -> cal sig_ksi_diff_tilt agent 2/4(ksi_diff_tilt_squ_gamma_2_2_vec)
  Constant33/1 -> Mux24/3
  Constant29/1 -> Mux26/2
  [sig_ksi_diff_tilt_gamma_1_node_4] -> combine sig_ksi_diff_tilt_gamma_1/4(sig_ksi_diff_tilt_gamma_1_node_4)
  cal abs 4/1(y) -> Mux24/1
  Constant98/1 -> Mux21/2
  cal high-order sliding mode differentiator position estimation error/1(ksi_diff_tilt_vec) -> [ksi_diff_tilt_vec]
  choose ksi_diff_tilt/1(y) -> cal abs 21/1(x)
  [ksi_diff_tilt_vec] -> choose ksi_diff_tilt 2/1(x)
  Mux7/1 -> Interpreted MATLAB Function8/1
  [ksi_diff_tilt_squ_1_2_vec] -> cal sig_ksi_diff_tilt agent 2/2(ksi_diff_tilt_squ_1_2_vec)
  [ksi_diff_tilt_vec] -> cal sig_ksi_diff_tilt agent 1/1(ksi_diff_tilt_vec)
  [ksi_diff_tilt_squ_gamma_2_2_node_3] -> combine ksi_diff_tilt_squ_gamma_2_2/3(ksi_diff_tilt_squ_gamma_2_2_node_3)
  Constant97/1 -> Mux22/3
  Interpreted MATLAB Function13/1 -> trans to column13/1(x)
  Mux25/1 -> Interpreted MATLAB Function4/1
  Constant50/1 -> Mux20/2
  Constant47/1 -> Mux19/2
  trans to column10/1(y) -> [ksi_diff_tilt_squ_1_2_node_4], Display11/1
  [sig_ksi_diff_tilt_1_2_node_5] -> combine sig_ksi_diff_tilt_1_2/5(sig_ksi_diff_tilt_1_2_node_5)
  [ksi_diff_tilt_vec] -> choose ksi_diff_tilt 4/1(x)
  Interpreted MATLAB Function8/1 -> trans to column8/1(x)
  choose ksi_diff_tilt3/1(y) -> cal abs 9/1(x)
  Constant26/1 -> Mux23/2
  Interpreted MATLAB Function4/1 -> trans to column4/1(x)
  cal abs 9/1(y) -> Mux12/1
  Mux24/1 -> Interpreted MATLAB Function3/1
  Interpreted MATLAB Function21/1 -> trans to column21/1(x)
  Constant45/1 -> Mux8/3
  [ksi_diff_tilt_squ_1_2_vec] -> cal sig_ksi_diff_tilt agent 5/2(ksi_diff_tilt_squ_1_2_vec)
  cal abs 1/1(y) -> Mux23/1
  [ksi_diff_tilt_vec] -> cal sig_ksi_diff_tilt agent 5/1(ksi_diff_tilt_vec)
  cal abs 11/1(y) -> Mux20/1
  Interpreted MATLAB Function10/1 -> trans to column10/1(x)
  [ksi_diff_tilt_squ_gamma_2_2_vec] -> cal sig_ksi_diff_tilt agent 5/4(ksi_diff_tilt_squ_gamma_2_2_vec)
  choose ksi_diff_tilt4/1(y) -> cal abs 13/1(x)
  [ksi_diff_tilt_squ_1_2_vec] -> cal sig_ksi_diff_tilt agent 4/2(ksi_diff_tilt_squ_1_2_vec)
  cal sig_ksi_diff_tilt agent 5/3(sig_ksi_diff_tilt_gamma_2_2_node_5) -> [sig_ksi_diff_tilt_gamma_2_2_node_5]
  Constant43/1 -> Mux12/3
  trans to column21/1(y) -> [ksi_diff_tilt_squ_1_2_node_1], Display51/1
  [ksi_diff_tilt_vec] -> cal sig_ksi_diff_tilt agent 4/1(ksi_diff_tilt_vec)
  trans to column20/1(y) -> [ksi_diff_tilt_squ_gamma_1_node_1], Display50/1
  cal abs 10/1(y) -> Mux8/1
  Constant30/1 -> Mux26/3
  Interpreted MATLAB Function2/1 -> trans to column2/1(x)
  [ksi_diff_tilt_vec] -> choose ksi_diff_tilt 9/1(x)
  [ksi_diff_tilt_squ_gamma_1_node_3] -> combine ksi_diff_tilt_squ_gamma_1/3(ksi_diff_tilt_squ_gamma_1_node_3)
  cal abs 12/1(y) -> Mux19/1
  Interpreted MATLAB Function20/1 -> trans to column20/1(x)
  Mux23/1 -> Interpreted MATLAB Function1/1
  Interpreted MATLAB Function12/1 -> trans to column12/1(x)
  [ksi_diff_tilt_squ_gamma_1_vec] -> cal sig_ksi_diff_tilt agent 4/3(ksi_diff_tilt_squ_gamma_1_vec)
  Constant28/1 -> Mux25/2
  [ksi_diff_tilt_vec] -> choose ksi_diff_tilt3/1(x)
  cal sig_ksi_diff_tilt agent 2/1(sig_ksi_diff_tilt_1_2_node_2) -> [sig_ksi_diff_tilt_1_2_node_2]
  [ksi_diff_tilt_vec] -> choose ksi_diff_tilt4/1(x)
  trans to column11/1(y) -> [ksi_diff_tilt_squ_1_2_node_5], Display27/1
  Constant46/1 -> Mux9/2
  cal abs 2/1(y) -> Mux26/1
  Constant27/1 -> Mux23/3
  Constant42/1 -> Mux7/3
  cal sig_ksi_diff_tilt agent 1/1(sig_ksi_diff_tilt_1_2_node_1) -> [sig_ksi_diff_tilt_1_2_node_1]
  [sig_ksi_diff_tilt_gamma_1_node_2] -> combine sig_ksi_diff_tilt_gamma_1/2(sig_ksi_diff_tilt_gamma_1_node_2)
  cal abs 21/1(y) -> Mux22/1
  [pos_diff_hat_vec] -> cal high-order sliding mode differentiator position estimation error/2(pos_diff_hat_vec)
  Mux19/1 -> Interpreted MATLAB Function12/1
  [ksi_diff_tilt_squ_gamma_1_vec] -> cal sig_ksi_diff_tilt agent 1/3(ksi_diff_tilt_squ_gamma_1_vec)
  [ksi_diff_tilt_vec] -> choose ksi_diff_tilt1/1(x)
  cal sig_ksi_diff_tilt agent 2/2(sig_ksi_diff_tilt_gamma_1_node_2) -> [sig_ksi_diff_tilt_gamma_1_node_2]
  Interpreted MATLAB Function9/1 -> trans to column9/1(x)
  cal sig_ksi_diff_tilt agent 5/1(sig_ksi_diff_tilt_1_2_node_5) -> [sig_ksi_diff_tilt_1_2_node_5]
  Mux20/1 -> Interpreted MATLAB Function13/1
  Constant49/1 -> Mux9/3
  cal abs 8/1(y) -> Mux7/1
  cal sig_ksi_diff_tilt agent 4/3(sig_ksi_diff_tilt_gamma_2_2_node_4) -> [sig_ksi_diff_tilt_gamma_2_2_node_4]
  [sig_ksi_diff_tilt_gamma_2_2_node_5] -> combine sig_ksi_diff_tilt_gamma_2_2/5(sig_ksi_diff_tilt_gamma_2_2_node_5)
  cal sig_ksi_diff_tilt agent 4/1(sig_ksi_diff_tilt_1_2_node_4) -> [sig_ksi_diff_tilt_1_2_node_4]
  combine sig_ksi_diff_tilt_gamma_1/1(sig_ksi_diff_tilt_gamma_1_vec) -> [sig_ksi_diff_tilt_gamma_1_vec]
  Interpreted MATLAB Function11/1 -> trans to column11/1(x)
  [sig_ksi_diff_tilt_gamma_1_node_5] -> combine sig_ksi_diff_tilt_gamma_1/5(sig_ksi_diff_tilt_gamma_1_node_5)
  [sig_ksi_diff_tilt_1_2_node_1] -> combine sig_ksi_diff_tilt_1_2/1(sig_ksi_diff_tilt_1_2_node_1)
  choose ksi_diff_tilt 4/1(y) -> cal abs 2/1(x)
  [sig_ksi_diff_tilt_gamma_2_2_node_3] -> combine sig_ksi_diff_tilt_gamma_2_2/3(sig_ksi_diff_tilt_gamma_2_2_node_3)
  Constant32/1 -> Mux24/2
  [ksi_diff_tilt_vec] -> choose ksi_diff_tilt 10/1(x)
  combine sig_ksi_diff_tilt_gamma_2_2/1(sig_ksi_diff_tilt_gamma_2_2_vec) -> [sig_ksi_diff_tilt_gamma_2_2_vec]
  [ksi_diff_tilt_squ_gamma_2_2_node_4] -> combine ksi_diff_tilt_squ_gamma_2_2/4(ksi_diff_tilt_squ_gamma_2_2_node_4)
  [ksi_diff_tilt_squ_gamma_2_2_vec] -> cal sig_ksi_diff_tilt agent 4/4(ksi_diff_tilt_squ_gamma_2_2_vec)
  Constant41/1 -> Mux7/2
  trans to column13/1(y) -> [ksi_diff_tilt_squ_gamma_1_node_5], Display26/1
  Mux12/1 -> Interpreted MATLAB Function10/1
  [sig_ksi_diff_tilt_gamma_2_2_node_2] -> combine sig_ksi_diff_tilt_gamma_2_2/2(sig_ksi_diff_tilt_gamma_2_2_node_2)
  Constant40/1 -> Mux12/2
  [ksi_diff_tilt_vec] -> choose ksi_diff_tilt 3/1(x)
  combine ksi_diff_tilt_squ_gamma_2_2/1(ksi_diff_tilt_squ_gamma_2_2_vec) -> [ksi_diff_tilt_squ_gamma_2_2_vec]
  [sig_ksi_diff_tilt_gamma_1_node_1] -> combine sig_ksi_diff_tilt_gamma_1/1(sig_ksi_diff_tilt_gamma_1_node_1)
  Mux8/1 -> Interpreted MATLAB Function9/1
  [d_vel_diff_hat_3] -> combine d_vel_diff_hat/3(d_vel_diff_hat_3)
  Constant62/1 -> cal vel_diff_hat agent 5/1(k_rho_1)
  [ksi_diff_tilt_vec] -> cal vel_diff_hat agent 5/7(ksi_diff_tilt_vec)
  [ksi_diff_tilt_vec] -> cal vel_diff_hat agent 4/7(ksi_diff_tilt_vec)
  Constant57/1 -> cal vel_diff_hat agent 4/1(k_rho_1)
  [sig_ksi_diff_tilt_gamma_1_vec] -> cal vel_diff_hat agent 4/8(sig_ksi_diff_tilt_gamma_1_vec)
  Constant65/1 -> cal vel_diff_hat agent 5/3(TTb)
  [tsim] -> cal vel_diff_hat agent 4/6(tsim)
  Constant59/1 -> cal vel_diff_hat agent 4/3(TTb)
  [tsim] -> cal vel_diff_hat agent 5/6(tsim)
  Constant60/1 -> cal vel_diff_hat agent 4/4(theta_1)
  vel_diff_hat Integrator 1/1 -> [vel_diff_hat_1]
  [tsim] -> cal vel_diff_hat agent 1/6(tsim)
  Constant63/1 -> cal vel_diff_hat agent 5/2(k_rho_2)
  cal vel_diff_hat agent 4/1(d_vel_diff_hat_4) -> vel_diff_hat Integrator 4/1, [d_vel_diff_hat_4]
  Constant61/1 -> cal vel_diff_hat agent 4/5(theta_2)
  combine vel_diff_hat/1(vel_diff_hat_vec) -> [vel_diff_hat_vec]
  Constant58/1 -> cal vel_diff_hat agent 4/2(k_rho_2)
  [d_vel_diff_hat_5] -> combine d_vel_diff_hat/5(d_vel_diff_hat_5)
  cal vel_diff_hat agent 5/1(d_vel_diff_hat_5) -> [d_vel_diff_hat_5], vel_diff_hat Integrator 5/1
  [vel_diff_hat_1] -> combine vel_diff_hat/1(vel_diff_hat_1)
  cal vel_diff_hat agent 2/1(d_vel_diff_hat_2) -> vel_diff_hat Integrator 2/1, [d_vel_diff_hat_2]
  [d_vel_diff_hat_2] -> combine d_vel_diff_hat/2(d_vel_diff_hat_2)
  Constant66/1 -> cal vel_diff_hat agent 5/4(theta_1)
  [vel_diff_hat_4] -> combine vel_diff_hat/4(vel_diff_hat_4)
  [d_vel_diff_hat_1] -> combine d_vel_diff_hat/1(d_vel_diff_hat_1)
  [ksi_diff_tilt_vec] -> cal vel_diff_hat agent 1/7(ksi_diff_tilt_vec)
  Constant67/1 -> cal vel_diff_hat agent 5/5(theta_2)
  [d_vel_diff_hat_4] -> combine d_vel_diff_hat/4(d_vel_diff_hat_4)
  Constant86/1 -> cal vel_diff_hat agent 1/1(k_rho_1)
  vel_diff_hat Integrator 5/1 -> [vel_diff_hat_5]
  [vel_diff_hat_3] -> combine vel_diff_hat/3(vel_diff_hat_3)
  [vel_diff_hat_2] -> combine vel_diff_hat/2(vel_diff_hat_2)
  Constant83/1 -> cal vel_diff_hat agent 2/4(theta_1)
  Constant90/1 -> cal vel_diff_hat agent 2/3(TTb)
  [tsim] -> cal vel_diff_hat agent 2/6(tsim)
  Constant53/1 -> cal vel_diff_hat agent 1/4(theta_1)
  [vel_diff_hat_5] -> combine vel_diff_hat/5(vel_diff_hat_5)
  [ksi_diff_tilt_vec] -> cal vel_diff_hat agent 2/7(ksi_diff_tilt_vec)
  [sig_ksi_diff_tilt_gamma_1_vec] -> cal vel_diff_hat agent 5/8(sig_ksi_diff_tilt_gamma_1_vec)
  Constant64/1 -> cal vel_diff_hat agent 1/5(theta_2)
  cal vel_diff_hat agent 1/1(d_vel_diff_hat_1) -> [d_vel_diff_hat_1], vel_diff_hat Integrator 1/1
  Constant84/1 -> cal vel_diff_hat agent 2/5(theta_2)
  Constant88/1 -> cal vel_diff_hat agent 1/3(TTb)
  Constant87/1 -> cal vel_diff_hat agent 1/2(k_rho_2)
  combine d_vel_diff_hat/1(d_vel_diff_hat_vec) -> [d_vel_diff_hat_vec]
  Constant85/1 -> cal vel_diff_hat agent 2/1(k_rho_1)
  vel_diff_hat Integrator 4/1 -> [vel_diff_hat_4]
  [sig_ksi_diff_tilt_gamma_1_vec] -> cal vel_diff_hat agent 2/8(sig_ksi_diff_tilt_gamma_1_vec)
  [sig_ksi_diff_tilt_gamma_1_vec] -> cal vel_diff_hat agent 1/8(sig_ksi_diff_tilt_gamma_1_vec)
  vel_diff_hat Integrator 2/1 -> [vel_diff_hat_2]
  Constant89/1 -> cal vel_diff_hat agent 2/2(k_rho_2)
  Constant73/1 -> cal pos_diff_hat agent 2/2(k_rho_2)
  [vel_diff_hat_vec] -> cal pos_diff_hat agent 5/7(vel_diff_hat_vec)
  cal pos_diff_hat agent 5/1(d_pos_diff_hat_5) -> pos_diff_hat Integrator 5/1
  Constant103/1 -> cal pos_diff_hat agent 5/5(theta_2)
  [sig_ksi_diff_tilt_gamma_2_2_vec] -> cal pos_diff_hat agent 5/9(sig_ksi_diff_tilt_gamma_2_2_vec)
  [tsim] -> cal pos_diff_hat agent 5/6(tsim)
  Constant82/1 -> cal pos_diff_hat agent 4/1(k_rho_1)
  [sig_ksi_diff_tilt_1_2_vec] -> cal pos_diff_hat agent 4/8(sig_ksi_diff_tilt_1_2_vec)
  Constant74/1 -> cal pos_diff_hat agent 2/3(TTb)
  Constant80/1 -> cal pos_diff_hat agent 4/4(theta_1)
  Constant71/1 -> cal pos_diff_hat agent 2/5(theta_2)
  Constant69/1 -> cal pos_diff_hat agent 1/5(theta_2)
  [sig_ksi_diff_tilt_1_2_vec] -> cal pos_diff_hat agent 5/8(sig_ksi_diff_tilt_1_2_vec)
  [sig_ksi_diff_tilt_1_2_vec] -> cal pos_diff_hat agent 2/8(sig_ksi_diff_tilt_1_2_vec)
  Constant105/1 -> cal pos_diff_hat agent 5/2(k_rho_2)
  Constant95/1 -> cal pos_diff_hat agent 1/2(k_rho_2)
  Constant101/1 -> cal pos_diff_hat agent 4/3(TTb)
  [tsim] -> cal pos_diff_hat agent 4/6(tsim)
  Constant93/1 -> cal pos_diff_hat agent 4/2(k_rho_2)
  cal pos_diff_hat agent 4/1(d_pos_diff_hat_4) -> pos_diff_hat Integrator 4/1
  [vel_diff_hat_vec] -> cal pos_diff_hat agent 4/7(vel_diff_hat_vec)
  [sig_ksi_diff_tilt_gamma_2_2_vec] -> cal pos_diff_hat agent 2/9(sig_ksi_diff_tilt_gamma_2_2_vec)
  [vel_diff_hat_vec] -> cal pos_diff_hat agent 2/7(vel_diff_hat_vec)
  Constant68/1 -> cal pos_diff_hat agent 1/4(theta_1)
  [sig_ksi_diff_tilt_1_2_vec] -> cal pos_diff_hat agent 1/8(sig_ksi_diff_tilt_1_2_vec)
  Constant106/1 -> cal pos_diff_hat agent 5/3(TTb)
  pos_diff_hat Integrator 1/1 -> [pos_diff_hat_1]
  Constant70/1 -> cal pos_diff_hat agent 2/4(theta_1)
  Constant96/1 -> cal pos_diff_hat agent 1/3(TTb)
  [pos_diff_hat_1] -> combine pos_diff_hat/1(pos_diff_hat_1)
  [pos_diff_hat_5] -> combine pos_diff_hat/5(pos_diff_hat_5)
  [pos_diff_hat_2] -> combine pos_diff_hat/2(pos_diff_hat_2)
  [tsim] -> cal pos_diff_hat agent 2/6(tsim)
  Constant94/1 -> cal pos_diff_hat agent 1/1(k_rho_1)
  pos_diff_hat Integrator 4/1 -> [pos_diff_hat_4]
  [sig_ksi_diff_tilt_gamma_2_2_vec] -> cal pos_diff_hat agent 1/9(sig_ksi_diff_tilt_gamma_2_2_vec)
  Constant102/1 -> cal pos_diff_hat agent 5/4(theta_1)
  combine pos_diff_hat/1(pos_diff_hat_vec) -> [pos_diff_hat_vec]
  cal pos_diff_hat agent 1/1(d_pos_diff_hat_1) -> pos_diff_hat Integrator 1/1
  [pos_diff_hat_4] -> combine pos_diff_hat/4(pos_diff_hat_4)
  Constant104/1 -> cal pos_diff_hat agent 5/1(k_rho_1)
  cal pos_diff_hat agent 2/1(d_pos_diff_hat_2) -> pos_diff_hat Integrator 2/1
  Constant72/1 -> cal pos_diff_hat agent 2/1(k_rho_1)
  [pos_diff_hat_3] -> combine pos_diff_hat/3(pos_diff_hat_3)
  [vel_diff_hat_vec] -> cal pos_diff_hat agent 1/7(vel_diff_hat_vec)
  [tsim] -> cal pos_diff_hat agent 1/6(tsim)
  Constant81/1 -> cal pos_diff_hat agent 4/5(theta_2)
  pos_diff_hat Integrator 2/1 -> [pos_diff_hat_2]
  pos_diff_hat Integrator 5/1 -> [pos_diff_hat_5]
  [sig_ksi_diff_tilt_gamma_2_2_vec] -> cal pos_diff_hat agent 4/9(sig_ksi_diff_tilt_gamma_2_2_vec)
  Demux36/3 -> Mux49/1
  Mux5/1 -> Scope4/1
  Demux37/1 -> Mux5/2
  Demux37/2 -> Mux6/2
  Mux17/1 -> Scope7/2
  [pos_diff_hat_vec] -> choose pos_diff_hat agent 2/1(x)
  Mux18/1 -> Scope7/3
  Mux16/1 -> Scope7/1
  Demux41/1 -> Mux28/2
  Demux6/2 -> Mux17/2
  [vel_diff_hat_vec] -> choose vel_diff_hat agent 2/1(x)
  Demux40/3 -> Mux30/1
  choose pos_diff_hat agent 1/1(y) -> Demux37/1
  Demux38/3 -> Mux15/1
  choose vel_diff_hat agent 1/1(y) -> Demux39/1
  Demux39/3 -> Mux15/2
  [vel_diff_hat_vec] -> choose vel_diff_hat agent 1/1(x)
  Mux6/1 -> Scope4/2
  choose ksi_i agent 1/1(y) -> Demux36/1
  choose eta_i agent 4/1(y) -> Demux17/1
  choose pos_diff_hat agent 5/1(y) -> Demux35/1
  Mux42/1 -> Scope10/3
  Mux14/1 -> Scope5/2
  Demux36/2 -> Mux6/1
  choose pos_diff_hat agent 3/1(y) -> Demux9/1
  Mux35/1 -> Scope8/2
  Demux6/3 -> Mux18/2
  choose eta_i agent 1/1(y) -> Demux38/1
  Demux17/3 -> Mux39/1
  Mux36/1 -> Scope8/3
  Demux38/2 -> Mux14/1
  Demux21/3 -> Mux45/1
  Demux8/1 -> Mux34/1
  Demux21/2 -> Mux44/1
  Demux10/3 -> Mux18/1
  Demux18/2 -> Mux38/2
  Demux37/3 -> Mux49/2
  Mux28/1 -> Scope6/1
  choose ksi_i agent 4/1(y) -> Demux19/1
  Demux18/3 -> Mux39/2
  Mux47/1 -> Scope12/2
  Demux20/1 -> Mux40/2
  choose eta_i agent 5/1(y) -> Demux21/1
  Mux38/1 -> Scope11/2
  Mux49/1 -> Scope4/3
  Mux43/1 -> Scope13/1
  Demux33/1 -> Mux43/2
  Mux33/1 -> Scope9/3
  Mux13/1 -> Scope5/1
  Mux44/1 -> Scope13/2
  Demux40/2 -> Mux29/1
  Demux33/2 -> Mux44/2
  Demux17/2 -> Mux38/1
  Demux19/2 -> Mux41/1
  Mux41/1 -> Scope10/2
  Demux20/2 -> Mux41/2
  Demux19/1 -> Mux40/1
  choose vel_diff_hat agent 4/1(y) -> Demux18/1
  Demux18/1 -> Mux37/2
  Demux19/3 -> Mux42/1
  Mux40/1 -> Scope10/1
  Demux40/1 -> Mux28/1
  Demux41/2 -> Mux29/2
  Demux17/1 -> Mux37/1
  choose pos_diff_hat agent 4/1(y) -> Demux20/1
  Demux12/3 -> Mux33/1
  choose ksi_i agent 2/1(y) -> Demux40/1
  Mux29/1 -> Scope6/2
  Demux7/2 -> Mux32/2
  [pos_diff_hat_vec] -> choose pos_diff_hat agent 3/1(x)
  Demux9/1 -> Mux34/2
  Demux36/1 -> Mux5/1
  Demux7/3 -> Mux33/2
  choose ksi_i agent 3/1(y) -> Demux8/1
  Demux7/1 -> Mux31/2
  Demux12/2 -> Mux32/1
  Demux41/3 -> Mux30/2
  Demux10/2 -> Mux17/1
  choose eta_i agent 2/1(y) -> Demux10/1
  Demux34/3 -> Mux48/1
  Mux32/1 -> Scope9/2
  [pos_diff_hat_vec] -> choose pos_diff_hat agent 1/1(x)
  [eta_i_vec] -> choose eta_i agent 2/1(x)
  Demux35/3 -> Mux48/2
  [vel_diff_hat_vec] -> choose vel_diff_hat agent 3/1(x)
  [eta_i_vec] -> choose eta_i agent 3/1(x)
  [vel_diff_hat_vec] -> choose vel_diff_hat agent 5/1(x)
  [eta_i_vec] -> choose eta_i agent 1/1(x)
  Mux39/1 -> Scope11/3
  choose pos_diff_hat agent 2/1(y) -> Demux41/1
  choose vel_diff_hat agent 2/1(y) -> Demux6/1
  Demux34/2 -> Mux47/1
  Mux31/1 -> Scope9/1
  Demux10/1 -> Mux16/1
  Demux39/1 -> Mux13/2
  choose eta_i agent 3/1(y) -> Demux12/1
  [ksi_i_vec] -> choose ksi_i agent 5/1(x)
  choose vel_diff_hat agent 3/1(y) -> Demux7/1
  Demux21/1 -> Mux43/1
  [eta_i_vec] -> choose eta_i agent 4/1(x)
  [ksi_i_vec] -> choose ksi_i agent 2/1(x)
  choose ksi_i agent 5/1(y) -> Demux34/1
  Demux12/1 -> Mux31/1
  Demux9/3 -> Mux36/2
  Demux38/1 -> Mux13/1
  Mux15/1 -> Scope5/3
  Mux46/1 -> Scope12/1
  Demux8/3 -> Mux36/1
  Demux39/2 -> Mux14/2
  Demux20/3 -> Mux42/2
  [eta_i_vec] -> choose eta_i agent 5/1(x)
  Mux30/1 -> Scope6/3
  [ksi_i_vec] -> choose ksi_i agent 4/1(x)
  [pos_diff_hat_vec] -> choose pos_diff_hat agent 4/1(x)
  Demux6/1 -> Mux16/2
  Demux34/1 -> Mux46/1
  Demux35/1 -> Mux46/2
  [ksi_i_vec] -> choose ksi_i agent 1/1(x)
  Mux34/1 -> Scope8/1
  [pos_diff_hat_vec] -> choose pos_diff_hat agent 5/1(x)
  [ksi_i_vec] -> choose ksi_i agent 3/1(x)
  Mux48/1 -> Scope12/3
  Mux45/1 -> Scope13/3
  Mux37/1 -> Scope11/1
  Demux8/2 -> Mux35/1
  choose vel_diff_hat agent 5/1(y) -> Demux33/1
  Demux9/2 -> Mux35/2
  Demux35/2 -> Mux47/2
  Demux33/3 -> Mux45/2
  [vel_diff_hat_vec] -> choose vel_diff_hat agent 4/1(x)
  choose ksi_diff_tilt 5/1(y) -> cal abs 7/1(x)
  choose ksi_diff_tilt 6/1(y) -> cal abs 5/1(x)
  trans to column5/1(y) -> [ksi_diff_tilt_squ_gamma_2_2_node_3], Display5/1
  cal sig_ksi_diff_tilt agent 3/2(sig_ksi_diff_tilt_gamma_1_node_3) -> [sig_ksi_diff_tilt_gamma_1_node_3]
  Constant34/1 -> Mux11/2
  cal sig_ksi_diff_tilt agent 3/1(sig_ksi_diff_tilt_1_2_node_3) -> [sig_ksi_diff_tilt_1_2_node_3]
  Mux11/1 -> Interpreted MATLAB Function7/1
  Interpreted MATLAB Function5/1 -> trans to column5/1(x)
  [ksi_diff_tilt_vec] -> choose ksi_diff_tilt 6/1(x)
  Interpreted MATLAB Function7/1 -> trans to column7/1(x)
  Mux10/1 -> Interpreted MATLAB Function6/1
  [ksi_diff_tilt_squ_1_2_vec] -> cal sig_ksi_diff_tilt agent 3/2(ksi_diff_tilt_squ_1_2_vec)
  Constant39/1 -> Mux10/3
  [ksi_diff_tilt_squ_gamma_1_vec] -> cal sig_ksi_diff_tilt agent 3/3(ksi_diff_tilt_squ_gamma_1_vec)
  cal sig_ksi_diff_tilt agent 3/3(sig_ksi_diff_tilt_gamma_2_2_node_3) -> [sig_ksi_diff_tilt_gamma_2_2_node_3]
  cal abs 6/1(y) -> Mux11/1
  Interpreted MATLAB Function6/1 -> trans to column6/1(x)
  Mux27/1 -> Interpreted MATLAB Function5/1
  [ksi_diff_tilt_vec] -> cal sig_ksi_diff_tilt agent 3/1(ksi_diff_tilt_vec)
  trans to column6/1(y) -> [ksi_diff_tilt_squ_gamma_1_node_3], Display7/1
  choose ksi_diff_tilt2/1(y) -> cal abs 6/1(x)
  Constant38/1 -> Mux10/2
  cal abs 7/1(y) -> Mux10/1
  Constant35/1 -> Mux27/2
  [ksi_diff_tilt_vec] -> choose ksi_diff_tilt 5/1(x)
  Constant37/1 -> Mux11/3
  Constant36/1 -> Mux27/3
  [ksi_diff_tilt_squ_gamma_2_2_vec] -> cal sig_ksi_diff_tilt agent 3/4(ksi_diff_tilt_squ_gamma_2_2_vec)
  trans to column7/1(y) -> [ksi_diff_tilt_squ_1_2_node_3], Display8/1
  cal abs 5/1(y) -> Mux27/1
  [ksi_diff_tilt_vec] -> choose ksi_diff_tilt2/1(x)
  Constant56/1 -> cal vel_diff_hat agent 3/1(k_rho_1)
  Constant91/1 -> cal vel_diff_hat agent 3/2(k_rho_2)
  vel_diff_hat Integrator 3/1 -> [vel_diff_hat_3]
  [ksi_diff_tilt_vec] -> cal vel_diff_hat agent 3/7(ksi_diff_tilt_vec)
  cal vel_diff_hat agent 3/1(d_vel_diff_hat_3) -> vel_diff_hat Integrator 3/1, [d_vel_diff_hat_3]
  Constant54/1 -> cal vel_diff_hat agent 3/4(theta_1)
  [sig_ksi_diff_tilt_gamma_1_vec] -> cal vel_diff_hat agent 3/8(sig_ksi_diff_tilt_gamma_1_vec)
  Constant55/1 -> cal vel_diff_hat agent 3/5(theta_2)
  [tsim] -> cal vel_diff_hat agent 3/6(tsim)
  Constant92/1 -> cal vel_diff_hat agent 3/3(TTb)
  pos_diff_hat Integrator 3/1 -> [pos_diff_hat_3]
  cal pos_diff_hat agent 3/1(d_pos_diff_hat_3) -> pos_diff_hat Integrator 3/1
  [sig_ksi_diff_tilt_gamma_2_2_vec] -> cal pos_diff_hat agent 3/9(sig_ksi_diff_tilt_gamma_2_2_vec)
  [sig_ksi_diff_tilt_1_2_vec] -> cal pos_diff_hat agent 3/8(sig_ksi_diff_tilt_1_2_vec)
  Constant76/1 -> cal pos_diff_hat agent 3/5(theta_2)
  Constant78/1 -> cal pos_diff_hat agent 3/2(k_rho_2)
  Constant79/1 -> cal pos_diff_hat agent 3/3(TTb)
  Constant77/1 -> cal pos_diff_hat agent 3/1(k_rho_1)
  Constant75/1 -> cal pos_diff_hat agent 3/4(theta_1)
  [tsim] -> cal pos_diff_hat agent 3/6(tsim)
  [vel_diff_hat_vec] -> cal pos_diff_hat agent 3/7(vel_diff_hat_vec)
  generate translational disturbance agent 5/1(dp_5) -> [dp_5]
  [dp_3] -> combine translational disturbance/3(dp_3)
  [dp_5] -> combine translational disturbance/5(dp_5)
  generate translational disturbance agent 4/1(dp_4) -> [dp_4]
  Constant286/1 -> generate translational disturbance agent 2/3(dp_phi_t)
  Constant295/1 -> generate translational disturbance agent 5/3(dp_phi_t)
  Constant107/1 -> generate translational disturbance agent 1/3(dp_phi_t)
  [dp_4] -> combine translational disturbance/4(dp_4)
  [tsim] -> generate translational disturbance agent 2/4(t)
  Constant287/1 -> generate translational disturbance agent 2/2(dp_ff_t)
  [tsim] -> generate translational disturbance agent 5/4(t)
  combine translational disturbance/1(dp_vec) -> [dp_vec]
  [tsim] -> generate translational disturbance agent 3/4(t)
  [dp_2] -> combine translational disturbance/2(dp_2)
  [dp_1] -> combine translational disturbance/1(dp_1)
  Constant285/1 -> generate translational disturbance agent 1/1(dp_aa_t)
  generate translational disturbance agent 1/1(dp_1) -> [dp_1]
  Constant108/1 -> generate translational disturbance agent 1/2(dp_ff_t)
  [tsim] -> generate translational disturbance agent 4/4(t)
  generate translational disturbance agent 2/1(dp_2) -> [dp_2]
  generate translational disturbance agent 3/1(dp_3) -> [dp_3]
  Constant289/1 -> generate translational disturbance agent 3/3(dp_phi_t)
  Constant294/1 -> generate translational disturbance agent 4/1(dp_aa_t)
  Constant296/1 -> generate translational disturbance agent 5/2(dp_ff_t)
  Constant292/1 -> generate translational disturbance agent 4/3(dp_phi_t)
  Constant291/1 -> generate translational disturbance agent 3/1(dp_aa_t)
  Constant290/1 -> generate translational disturbance agent 3/2(dp_ff_t)
  Constant297/1 -> generate translational disturbance agent 5/1(dp_aa_t)
  Constant293/1 -> generate translational disturbance agent 4/2(dp_ff_t)
  [tsim] -> generate translational disturbance agent 1/4(t)
  Constant288/1 -> generate translational disturbance agent 2/1(dp_aa_t)
  [ksi_est_err] -> To Workspace17/1
  [eta_est_err] -> To Workspace22/1
  [ksi_d_est_vec] -> To Workspace18/1
  [sigma_v_vec] -> To Workspace19/1
  [eta_i_vec] -> To Workspace7/1
  [eta_d_est_vec] -> To Workspace/1
  [ksi_track_err_vec] -> To Workspace9/1
  [eta0] -> To Workspace4/1
  [ui] -> To Workspace14/1
  [ksi_i_vec] -> To Workspace8/1
  [eta_track_err_vec] -> To Workspace10/1
  [sigma_bar_v_tilt_vec] -> To Workspace13/1
  [ksi0] -> To Workspace5/1
  [dp_vec] -> To Workspace2/1
  [sigma_bar_v_hat_vec] -> To Workspace11/1
  [dp_hat_vec] -> To Workspace1/1
  [u0] -> To Workspace3/1
  [vel_diff_hat_vec] -> To Workspace20/1
  [sigma_bar_v_vec] -> To Workspace12/1
  [pos_diff_hat_vec] -> To Workspace21/1
  [dp_tilt_vec] -> To Workspace6/1
  [eta0] -> desire formation position and velocity/2(eta0)
  process velocity/1(V_init_out) -> [V_init_out]
  set desire formation configuration/3(d_delta_eta_vec) -> [d_delta_eta_vec]
  Constant/1 -> leader control input/2(T1)
  Constant114/1 -> process velocity/8(Rx2)
  [ksi0] -> desire formation position and velocity/1(ksi0)
  Constant226/1 -> set desire formation configuration/9(Z3)
  desire formation position and velocity/2(vel_i_des) -> [vel_i_des]
  leader ksi0 Integrator/1 -> [ksi0]
  [tsim] -> process velocity/11(t)
  Constant231/1 -> set desire formation configuration/11(kai_1_t)
  Constant127/1 -> process velocity/4(PZ0)
  [delta_ksi_vec] -> desire formation position and velocity/3(delta_ksi_vec)
  Constant112/1 -> process velocity/10(Rz2)
  Demux22/1 -> eta_0/1
  Constant234/1 -> set desire formation configuration/3(X3)
  Constant117/1 -> set desire formation configuration/4(Y1)
  Clock/1 -> [tsim]
  set desire formation configuration/1(delta_ksi_vec) -> [delta_ksi_vec]
  [tsim] -> leader control input/1(t)
  Constant122/1 -> leader control input/6(Rx2)
  Constant235/1 -> set desire formation configuration/12(kai_3_t)
  [delta_eta_vec] -> desire formation position and velocity/4(delta_eta_vec)
  [eta0] -> Demux22/1
  set desire formation configuration/2(delta_eta_vec) -> [delta_eta_vec]
  Demux1/3 -> ksi_0/3
  leader eta0 Integrator/1 -> [eta0], leader ksi0 Integrator/1
  leader control input/1(u0) -> [u0]
  [ksi0] -> Demux1/1
  Constant222/1 -> set desire formation configuration/8(Z2)
  Constant124/1 -> leader control input/8(Rz2)
  [u0] -> leader eta0 Integrator/1
  Constant116/1 -> set desire formation configuration/2(X2)
  Constant238/1 -> set desire formation configuration/13(T1)
  Constant111/1 -> process velocity/1(T0)
  Step/1 -> leader eta0 Integrator/2
  [tsim] -> set desire formation configuration/15(t)
  desire formation position and velocity/1(pos_i_des) -> [pos_i_des]
  Constant115/1 -> set desire formation configuration/1(X1)
  Constant119/1 -> leader control input/3(T2)
  Constant121/1 -> leader control input/5(R1)
  Constant126/1 -> process velocity/2(T1)
  Constant125/1 -> process velocity/3(T2)
  Constant221/1 -> set desire formation configuration/7(Z1)
  Constant118/1 -> set desire formation configuration/5(Y2)
  Constant239/1 -> set desire formation configuration/14(T12)
  Constant110/1 -> process velocity/7(R1)
  Constant229/1 -> set desire formation configuration/6(Y3)
  Constant120/1 -> leader control input/4(R0)
  Constant109/1 -> process velocity/6(R0)
  Constant123/1 -> leader control input/7(Ry2)
  [V_init_out] -> leader eta0 Integrator/3
  Demux22/2 -> eta_0/2
  Constant128/1 -> process velocity/5(PZ1)
  Constant113/1 -> process velocity/9(Ry2)
  Demux1/2 -> ksi_0/2
  Constant225/1 -> set desire formation configuration/10(theta0)
  Demux1/1 -> ksi_0/1
  Demux22/3 -> eta_0/3
  [delta_ksi_vec] -> follower tracking error agent 1/1(delta_ksi_vec)
  [delta_eta_vec] -> follower tracking error agent 1/2(delta_eta_vec)
  [delta_eta_vec] -> follower tracking error agent 2/2(delta_eta_vec)
  [delta_ksi_vec] -> follower tracking error agent 2/1(delta_ksi_vec)
  [delta_eta_vec] -> follower tracking error agent 3/2(delta_eta_vec)
  [delta_ksi_vec] -> follower tracking error agent 3/1(delta_ksi_vec)
  [delta_eta_vec] -> follower tracking error agent 4/2(delta_eta_vec)
  [delta_ksi_vec] -> follower tracking error agent 4/1(delta_ksi_vec)
  [delta_eta_vec] -> follower tracking error agent 5/2(delta_eta_vec)
  [delta_ksi_vec] -> follower tracking error agent 5/1(delta_ksi_vec)
  fixed-time distributed follower desire position observer agent 4/1(d_ksi_d_est_4) -> position observe Integrator 4/1
  [theta_ksi_est_err_tilt_1_5] -> combine lumped follower position observation error/5(theta_ksi_est_err_tilt_1_5)
  Constant256/1 -> Mux112/2
  [theta_eta_est_err_tilt_2_vec] -> fixed-time distributed follower desire velocity observer agent 5/4(theta_eta_est_err_tilt_2_vec)
  [ksi_d_est_4] -> combine leader position estimaters/4(ksi_d_est_4)
  trans to column45/1(y) -> [ksi_est_err_squ_1_node_1], Display84/1
  Mux86/1 -> ksi_d_est_1/1
  trans to column50/1(y) -> [ksi_est_err_squ_2_node_5], Display85/1
  [theta_ksi_est_err_tilt_1_1] -> combine lumped follower position observation error/1(theta_ksi_est_err_tilt_1_1)
  Mux129/1 -> Interpreted MATLAB Function51/1
  Constant281/1 -> Mux128/2
  Mux88/1 -> ksi_d_est_4/2
  [eta_est_err_tilt_vec] -> choose eta_est_err_tilt 10/1(x)
  Add5/1 -> Demux88/1
  Demux78/1 -> Mux86/1
  Constant283/1 -> cal theta_ksi_est_err_tilt agent 1/1(alfa_theta)
  Constant252/1 -> fixed-time distributed follower desire position observer agent 3/2(l2p)
  Constant248/1 -> Mux109/3
  Mux112/1 -> Interpreted MATLAB Function55/1
  Add/1 -> Demux70/1
  Mux134/1 -> ksi_d_est_3/2
  cal abs 55/1(y) -> Mux110/1
  Constant255/1 -> Mux113/3
  Mux128/1 -> Interpreted MATLAB Function50/1
  [theta_ksi_est_err_tilt_2_4] -> combine lumped follower position observation error/9(theta_ksi_est_err_tilt_2_4)
  choose eta_est_err_tilt 13/1(y) -> cal abs 45/1(x)
  cal abs 51/1(y) -> Mux125/1
  Mux114/1 -> Interpreted MATLAB Function57/1
  Constant262/1 -> Mux118/2
  Interpreted MATLAB Function56/1 -> trans to column56/1(x)
  Demux75/1 -> Mux102/1
  cal theta_eta_est_err_tilt agent 4/1(theta_eta_est_err_tilt_1_4) -> [theta_eta_est_err_tilt_1_4]
  trans to column51/1(y) -> [ksi_est_err_squ_1_node_5], Display86/1
  Mux130/1 -> ksi_d_est_2/2
  Demux72/1 -> Mux95/2
  [ksi_est_err_squ_1_node_1] -> cal theta_ksi_est_err_tilt agent 1/2(ksi_est_err_squ_1_node_1)
  Constant185/1 -> cal theta_ksi_est_err_tilt agent 4/1(alfa_theta)
  [theta_eta_est_err_tilt_1_3] -> combine lumped follower velocity observation error/3(theta_eta_est_err_tilt_1_3)
  Mux93/1 -> eta_d_est_1/2
  Demux73/2 -> Mux100/1
  Mux132/1 -> ksi_d_est_2/3
  Interpreted MATLAB Function48/1 -> trans to column48/1(x)
  Mux102/1 -> eta_d_est_4/1
  [ksi_est_err_tilt_vec] -> choose eta_est_err_tilt 14/1(x)
  cal abs 52/1(y) -> Mux109/1
  [theta_eta_est_err_tilt_1_vec] -> fixed-time distributed follower desire velocity observer agent 4/3(theta_eta_est_err_tilt_1_vec)
  [eta0] -> Add2/1
  velocity observe Integrator 2/1 -> [eta_d_est_2], Demux71/1
  [ksi_est_err_tilt_vec] -> cal theta_ksi_est_err_tilt agent 3/4(ksi_est_err_tilt_vec)
  [ksi_est_err_tilt_vec] -> cal theta_ksi_est_err_tilt agent 5/4(ksi_est_err_tilt_vec)
  Mux124/1 -> Interpreted MATLAB Function47/1
  trans to column58/1(y) -> [eta_est_err_squ_1_node_4], Display92/1
  Constant269/1 -> Mux121/3
  [ksi_d_est_2] -> combine leader position estimaters/2(ksi_d_est_2)
  [eta_d_est_vec] -> fixed-time distributed follower desire position observer agent 4/3(eta_d_est_vec)
  combine leader position estimaters/1(ksi_d_est_vec) -> [ksi_d_est_vec]
  Mux92/1 -> eta_d_est_1/1
  [theta_eta_est_err_tilt_1_5] -> combine lumped follower velocity observation error/5(theta_eta_est_err_tilt_1_5)
  cal theta_eta_est_err_tilt agent 1/1(theta_eta_est_err_tilt_1_1) -> [theta_eta_est_err_tilt_1_1]
  Constant190/1 -> fixed-time distributed follower desire position observer agent 5/1(l1p)
  Demux95/3 -> Mux135/2
  Constant246/1 -> Mux115/3
  fixed-time distributed follower desire position observer agent 3/1(d_ksi_d_est_3) -> position observe Integrator 3/1
  [eta_est_err_tilt_vec] -> choose eta_est_err_tilt 9/1(x)
  [eta_est_err_tilt_vec] -> cal theta_eta_est_err_tilt agent 1/4(eta_est_err_tilt_vec)
  [ksi_est_err_tilt_vec] -> choose eta_est_err_tilt 13/1(x)
  Demux74/1 -> Mux99/2
  Constant209/1 -> fixed-time distributed follower desire velocity observer agent 4/2(l2v)
  Demux75/2 -> Mux103/1
  Demux70/3 -> Mux94/2
  Demux93/1 -> Mux119/2
  cal theta_ksi_est_err_tilt agent 1/2(theta_ksi_est_err_tilt_2_1) -> [theta_ksi_est_err_tilt_2_1]
  Constant271/1 -> Mux124/3
  choose eta_est_err_tilt 3/1(y) -> cal abs 54/1(x)
  [eta0] -> Add1/1
  [ksi_est_err_tilt_vec] -> choose eta_est_err_tilt 15/1(x)
  Demux79/1 -> Mux105/2
  Constant217/1 -> Mux120/2
  Constant241/1 -> Add6/2
  trans to column60/1(y) -> [eta_est_err_squ_1_node_5], Display95/1
  Constant183/1 -> fixed-time distributed follower desire position observer agent 4/2(l2p)
  Demux96/3 -> Mux89/1
  fixed-time distributed follower desire velocity observer agent 3/1(d_eta_d_est_3) -> velocity observe Integrator 3/1
  Demux75/3 -> Mux104/1
  Demux97/1 -> Mux87/2
  [eta0] -> Add4/1
  choose eta_est_err_tilt 15/1(y) -> cal abs 47/1(x)
  Demux70/1 -> Mux92/2
  Demux96/2 -> Mux88/1
  [eta_est_err_squ_2_node_2] -> cal theta_eta_est_err_tilt agent 2/3(eta_est_err_squ_2_node_2)
  Add3/1 -> Demux76/1
  Add7/1 -> Demux95/1
  Constant211/1 -> Add3/2
  [eta_est_err_tilt_vec] -> cal theta_eta_est_err_tilt agent 2/4(eta_est_err_tilt_vec)
  Demux71/3 -> Mux98/1
  [eta_est_err_squ_1_node_5] -> cal theta_eta_est_err_tilt agent 5/2(eta_est_err_squ_1_node_5)
  [ksi0] -> Add8/1
  Mux117/1 -> Interpreted MATLAB Function59/1
  cal theta_eta_est_err_tilt agent 5/2(theta_eta_est_err_tilt_2_5) -> [theta_eta_est_err_tilt_2_5]
  Demux74/2 -> Mux100/2
  Demux80/1 -> Mux90/2
  Constant201/1 -> Add/2
  cal theta_eta_est_err_tilt agent 2/1(theta_eta_est_err_tilt_1_2) -> [theta_eta_est_err_tilt_1_2]
  Demux76/2 -> Mux103/2
  cal abs 54/1(y) -> Mux111/1
  Constant263/1 -> fixed-time distributed follower desire position observer agent 3/1(l1p)
  Mux133/1 -> ksi_d_est_3/1
  [eta_d_est_3] -> combine follower desire velocity estimaters/3(eta_d_est_3)
  combine lumped follower velocity observation error/1(theta_eta_est_err_tilt_1_vec) -> [theta_eta_est_err_tilt_1_vec]
  Interpreted MATLAB Function46/1 -> trans to column46/1(x)
  trans to column48/1(y) -> [ksi_est_err_squ_2_node_4], Display82/1
  Mux118/1 -> Interpreted MATLAB Function60/1
  Mux101/1 -> eta_d_est_3/3
  combine lumped follower position observation error/1(theta_ksi_est_err_tilt_1_vec) -> [theta_ksi_est_err_tilt_1_vec]
  [theta_eta_est_err_tilt_1_vec] -> fixed-time distributed follower desire velocity observer agent 1/3(theta_eta_est_err_tilt_1_vec)
  Constant260/1 -> Mux114/2
  Constant230/1 -> fixed-time distributed follower desire position observer agent 2/1(l1p)
  Demux68/3 -> Mux131/1
  Add4/1 -> Demux79/1
  [ksi_est_err_tilt_vec] -> cal theta_ksi_est_err_tilt agent 4/4(ksi_est_err_tilt_vec)
  fixed-time distributed follower desire velocity observer agent 1/1(d_eta_d_est_1) -> velocity observe Integrator 1/1
  [ksi_est_err_squ_2_node_1] -> cal theta_ksi_est_err_tilt agent 1/3(ksi_est_err_squ_2_node_1)
  Constant276/1 -> Mux127/3
  trans to column43/1(y) -> [ksi_est_err_squ_2_node_2], Display78/1
  [eta_d_est_vec] -> fixed-time distributed follower desire position observer agent 3/3(eta_d_est_vec)
  Interpreted MATLAB Function47/1 -> trans to column47/1(x)
  Interpreted MATLAB Function43/1 -> trans to column43/1(x)
  choose eta_est_err_tilt 11/1(y) -> cal abs 43/1(x)
  Demux73/1 -> Mux99/1
  [eta_est_err_tilt_vec] -> cal theta_eta_est_err_tilt agent 5/4(eta_est_err_tilt_vec)
  Mux89/1 -> ksi_d_est_4/3
  [ksi0] -> Add5/1
  Constant195/1 -> cal theta_eta_est_err_tilt agent 3/1(alfa_theta)
  choose eta_est_err_tilt 12/1(y) -> cal abs 44/1(x)
  combine lumped follower velocity observation error/2(theta_eta_est_err_tilt_2_vec) -> [theta_eta_est_err_tilt_2_vec]
  [theta_eta_est_err_tilt_2_1] -> combine lumped follower velocity observation error/6(theta_eta_est_err_tilt_2_1)
  Demux71/2 -> Mux96/1
  Mux106/1 -> eta_d_est_5/2
  cal abs 41/1(y) -> Mux115/1
  Constant264/1 -> Mux118/3
  Mux126/1 -> Interpreted MATLAB Function45/1
  [eta_d_est_5] -> combine follower desire velocity estimaters/5(eta_d_est_5)
  Demux70/2 -> Mux93/2
  Interpreted MATLAB Function57/1 -> trans to column57/1(x)
  Demux94/1 -> Mux133/1
  Constant215/1 -> Mux126/2
  velocity observe Integrator 3/1 -> [eta_d_est_3], Demux73/1
  cal abs 44/1(y) -> Mux128/1
  Demux77/2 -> Mux106/1
  Mux115/1 -> Interpreted MATLAB Function54/1
  [ksi_est_err_tilt_vec] -> choose eta_est_err_tilt 18/1(x)
  [theta_ksi_est_err_tilt_2_3] -> combine lumped follower position observation error/8(theta_ksi_est_err_tilt_2_3)
  Demux74/3 -> Mux101/2
  cal abs 43/1(y) -> Mux126/1
  [theta_eta_est_err_tilt_2_5] -> combine lumped follower velocity observation error/10(theta_eta_est_err_tilt_2_5)
  Mux91/1 -> ksi_d_est_5/2
  cal abs 59/1(y) -> Mux114/1
  [ksi_est_err_tilt_vec] -> cal theta_ksi_est_err_tilt agent 1/4(ksi_est_err_tilt_vec)
  Constant199/1 -> fixed-time distributed follower desire velocity observer agent 1/2(l2v)
  [theta_eta_est_err_tilt_2_vec] -> fixed-time distributed follower desire velocity observer agent 1/4(theta_eta_est_err_tilt_2_vec)
  [theta_ksi_est_err_tilt_2_vec] -> fixed-time distributed follower desire position observer agent 2/5(theta_ksi_est_err_tilt_2_vec)
  Constant257/1 -> Mux112/3
  [eta_est_err_tilt_vec] -> choose eta_est_err_tilt 7/1(x)
  Constant274/1 -> Add7/2
  [theta_eta_est_err_tilt_1_vec] -> fixed-time distributed follower desire velocity observer agent 5/3(theta_eta_est_err_tilt_1_vec)
  [ksi_est_err_squ_1_node_5] -> cal theta_ksi_est_err_tilt agent 5/2(ksi_est_err_squ_1_node_5)
  [theta_ksi_est_err_tilt_1_2] -> combine lumped follower position observation error/2(theta_ksi_est_err_tilt_1_2)
  choose eta_est_err_tilt 17/1(y) -> cal abs 49/1(x)
  Demux77/3 -> Mux107/1
  trans to column52/1(y) -> [eta_est_err_squ_2_node_2], Display87/1
  Mux131/1 -> ksi_d_est_5/3
  choose eta_est_err_tilt 20/1(y) -> cal abs 53/1(x)
  [eta_est_err_tilt_vec] -> choose eta_est_err_tilt 3/1(x)
  [ksi0] -> Add6/1
  choose eta_est_err_tilt 2/1(y) -> cal abs 52/1(x)
  cal theta_ksi_est_err_tilt agent 5/2(theta_ksi_est_err_tilt_2_5) -> [theta_ksi_est_err_tilt_2_5]
  trans to column42/1(y) -> [ksi_est_err_squ_2_node_1], Display77/1
  Interpreted MATLAB Function44/1 -> trans to column44/1(x)
  fixed-time distributed follower desire position observer agent 2/1(d_ksi_d_est_2) -> position observe Integrator 2/1
  [eta_est_err_squ_2_node_3] -> cal theta_eta_est_err_tilt agent 3/3(eta_est_err_squ_2_node_3)
  Demux95/1 -> Mux133/2
  cal abs 47/1(y) -> Mux121/1
  [ksi_est_err_squ_2_node_2] -> cal theta_ksi_est_err_tilt agent 2/3(ksi_est_err_squ_2_node_2)
  Constant249/1 -> Mux111/2
  Demux77/1 -> Mux105/1
  [ksi_d_est_1] -> combine leader position estimaters/1(ksi_d_est_1)
  Constant251/1 -> Mux110/2
  [theta_ksi_est_err_tilt_2_1] -> combine lumped follower position observation error/6(theta_ksi_est_err_tilt_2_1)
  Constant189/1 -> fixed-time distributed follower desire position observer agent 5/2(l2p)
  Mux125/1 -> Interpreted MATLAB Function48/1
  Demux69/3 -> Mux94/1
  Constant277/1 -> Mux125/2
  Mux108/1 -> ksi_d_est_1/3
  Mux105/1 -> eta_d_est_5/1
  Constant188/1 -> Add8/2
  [eta_d_est_vec] -> fixed-time distributed follower desire position observer agent 1/3(eta_d_est_vec)
  Demux92/3 -> Mux132/1
  [ksi_est_err_tilt_vec] -> choose eta_est_err_tilt 17/1(x)
  Add9/1 -> Demux80/1
  Constant253/1 -> Mux110/3
  choose eta_est_err_tilt 4/1(y) -> cal abs 55/1(x)
  Add6/1 -> Demux93/1
  combine lumped follower position observation error/2(theta_ksi_est_err_tilt_2_vec) -> [theta_ksi_est_err_tilt_2_vec]
  [eta_est_err_squ_1_node_4] -> cal theta_eta_est_err_tilt agent 4/2(eta_est_err_squ_1_node_4)
  position observe Integrator 1/1 -> [ksi_d_est_1], Demux78/1
  [eta_est_err_tilt_vec] -> choose eta_est_err_tilt 6/1(x)
  Constant182/1 -> fixed-time distributed follower desire position observer agent 1/2(l2p)
  Demux88/2 -> Mux97/2
  choose eta_est_err_tilt 8/1(y) -> cal abs 59/1(x)
  Constant278/1 -> Mux125/3
  [theta_ksi_est_err_tilt_1_3] -> combine lumped follower position observation error/3(theta_ksi_est_err_tilt_1_3)
  cal theta_ksi_est_err_tilt agent 2/1(theta_ksi_est_err_tilt_1_2) -> [theta_ksi_est_err_tilt_1_2]
  Constant254/1 -> Mux113/2
  velocity observe Integrator 1/1 -> [eta_d_est_1], Demux69/1
  Constant282/1 -> Mux128/3
  fixed-time distributed follower desire velocity observer agent 5/1(d_eta_d_est_5) -> velocity observe Integrator 5/1
  position observe Integrator 5/1 -> [ksi_d_est_5], Demux68/1
  Demux78/3 -> Mux108/1
  choose eta_est_err_tilt 7/1(y) -> cal abs 58/1(x)
  Mux107/1 -> eta_d_est_5/3
  choose eta_est_err_tilt 10/1(y) -> cal abs 42/1(x)
  Constant197/1 -> fixed-time distributed follower desire position observer agent 1/1(l1p)
  choose eta_est_err_tilt 5/1(y) -> cal abs 56/1(x)
  [eta_est_err_squ_2_node_4] -> cal theta_eta_est_err_tilt agent 4/3(eta_est_err_squ_2_node_4)
  [theta_eta_est_err_tilt_2_vec] -> fixed-time distributed follower desire velocity observer agent 2/4(theta_eta_est_err_tilt_2_vec)
  Demux78/2 -> Mux97/1
  [theta_eta_est_err_tilt_1_vec] -> fixed-time distributed follower desire velocity observer agent 2/3(theta_eta_est_err_tilt_1_vec)
  choose eta_est_err_tilt 19/1(y) -> cal abs 51/1(x)
  Constant196/1 -> cal theta_eta_est_err_tilt agent 4/1(alfa_theta)
  Interpreted MATLAB Function58/1 -> trans to column58/1(x)
  Constant200/1 -> fixed-time distributed follower desire velocity observer agent 1/1(l1v)
  [ksi_est_err_tilt_vec] -> choose eta_est_err_tilt 20/1(x)
  Demux80/3 -> Mux131/2
  Mux135/1 -> ksi_d_est_3/3
  Constant250/1 -> Mux111/3
  cal theta_eta_est_err_tilt agent 4/2(theta_eta_est_err_tilt_2_4) -> [theta_eta_est_err_tilt_2_4]
  Add1/1 -> Demux72/1
  Demux68/1 -> Mux90/1
  Add2/1 -> Demux74/1
  [ksi_est_err_squ_2_node_5] -> cal theta_ksi_est_err_tilt agent 5/3(ksi_est_err_squ_2_node_5)
  cal theta_ksi_est_err_tilt agent 5/1(theta_ksi_est_err_tilt_1_5) -> [theta_ksi_est_err_tilt_1_5]
  [ksi_est_err_squ_1_node_2] -> cal theta_ksi_est_err_tilt agent 2/2(ksi_est_err_squ_1_node_2)
  cal abs 50/1(y) -> Mux127/1
  [ksi_est_err_squ_1_node_4] -> cal theta_ksi_est_err_tilt agent 4/2(ksi_est_err_squ_1_node_4)
  [theta_ksi_est_err_tilt_1_vec] -> fixed-time distributed follower desire position observer agent 4/4(theta_ksi_est_err_tilt_1_vec)
  Demux76/3 -> Mux104/2
  [eta_est_err_tilt_vec] -> choose eta_est_err_tilt 5/1(x)
  Interpreted MATLAB Function53/1 -> trans to column53/1(x)
  Demux88/3 -> Mux108/2
  position observe Integrator 3/1 -> [ksi_d_est_3], Demux94/1
  [theta_ksi_est_err_tilt_2_2] -> combine lumped follower position observation error/7(theta_ksi_est_err_tilt_2_2)
  Constant210/1 -> fixed-time distributed follower desire velocity observer agent 4/1(l1v)
  Mux111/1 -> Interpreted MATLAB Function53/1
  [eta0] -> Add3/1
  Demux88/1 -> Mux86/2
  cal theta_eta_est_err_tilt agent 2/2(theta_eta_est_err_tilt_2_2) -> [theta_eta_est_err_tilt_2_2]
  Constant267/1 -> Mux122/3
  Constant275/1 -> Mux127/2
  Interpreted MATLAB Function50/1 -> trans to column50/1(x)
  [ksi_est_err_tilt_vec] -> choose eta_est_err_tilt 12/1(x)
  velocity observe Integrator 4/1 -> [eta_d_est_4], Demux75/1
  cal theta_eta_est_err_tilt agent 1/2(theta_eta_est_err_tilt_2_1) -> [theta_eta_est_err_tilt_2_1]
  Mux110/1 -> Interpreted MATLAB Function52/1
  [ksi_est_err_tilt_vec] -> choose eta_est_err_tilt 11/1(x)
  [eta_d_est_vec] -> fixed-time distributed follower desire position observer agent 5/3(eta_d_est_vec)
  Constant204/1 -> Add1/2
  cal abs 56/1(y) -> Mux113/1
  cal theta_ksi_est_err_tilt agent 3/2(theta_ksi_est_err_tilt_2_3) -> [theta_ksi_est_err_tilt_2_3]
  [eta_est_err_tilt_vec] -> choose eta_est_err_tilt 4/1(x)
  Mux97/1 -> ksi_d_est_1/2
  cal theta_ksi_est_err_tilt agent 4/2(theta_ksi_est_err_tilt_2_4) -> [theta_ksi_est_err_tilt_2_4]
  [theta_ksi_est_err_tilt_1_vec] -> fixed-time distributed follower desire position observer agent 3/4(theta_ksi_est_err_tilt_1_vec)
  [eta_d_est_vec] -> fixed-time distributed follower desire position observer agent 2/3(eta_d_est_vec)
  trans to column55/1(y) -> [eta_est_err_squ_2_node_3], Display89/1
  velocity observe Integrator 5/1 -> [eta_d_est_5], Demux77/1
  Constant213/1 -> fixed-time distributed follower desire velocity observer agent 5/1(l1v)
  Interpreted MATLAB Function55/1 -> trans to column55/1(x)
  cal abs 53/1(y) -> Mux129/1
  Demux73/3 -> Mux101/1
  [ksi_est_err_squ_2_node_4] -> cal theta_ksi_est_err_tilt agent 4/3(ksi_est_err_squ_2_node_4)
  Mux99/1 -> eta_d_est_3/1
  trans to column49/1(y) -> [ksi_est_err_squ_1_node_4], Display83/1
  position observe Integrator 2/1 -> [ksi_d_est_2], Demux92/1
  trans to column54/1(y) -> [eta_est_err_squ_1_node_1], Display93/1
  trans to column47/1(y) -> [ksi_est_err_squ_1_node_3], Display81/1
  [theta_ksi_est_err_tilt_2_vec] -> fixed-time distributed follower desire position observer agent 4/5(theta_ksi_est_err_tilt_2_vec)
  cal theta_ksi_est_err_tilt agent 1/1(theta_ksi_est_err_tilt_1_1) -> [theta_ksi_est_err_tilt_1_1]
  Demux95/2 -> Mux134/2
  Constant265/1 -> Mux117/2
  trans to column53/1(y) -> [eta_est_err_squ_1_node_2], Display88/1
  Constant284/1 -> cal theta_ksi_est_err_tilt agent 2/1(alfa_theta)
  Constant216/1 -> Mux126/3
  [ksi_est_err_squ_2_node_3] -> cal theta_ksi_est_err_tilt agent 3/3(ksi_est_err_squ_2_node_3)
  Demux97/2 -> Mux88/2
  Mux109/1 -> Interpreted MATLAB Function41/1
  Constant218/1 -> Mux120/3
  Demux93/2 -> Mux130/2
  Interpreted MATLAB Function52/1 -> trans to column52/1(x)
  Demux71/1 -> Mux95/1
  Constant245/1 -> Mux115/2
  cal abs 42/1(y) -> Mux117/1
  Constant212/1 -> fixed-time distributed follower desire velocity observer agent 5/2(l2v)
  fixed-time distributed follower desire position observer agent 5/1(d_ksi_d_est_5) -> position observe Integrator 5/1
  Demux69/2 -> Mux93/1
  Mux123/1 -> Interpreted MATLAB Function46/1
  [theta_eta_est_err_tilt_1_4] -> combine lumped follower velocity observation error/4(theta_eta_est_err_tilt_1_4)
  Interpreted MATLAB Function41/1 -> trans to column41/1(x)
  [theta_eta_est_err_tilt_2_4] -> combine lumped follower velocity observation error/9(theta_eta_est_err_tilt_2_4)
  Constant258/1 -> Mux116/2
  Interpreted MATLAB Function42/1 -> trans to column42/1(x)
  Mux116/1 -> Interpreted MATLAB Function58/1
  Mux96/1 -> eta_d_est_2/2
  [ksi_est_err_tilt_vec] -> cal theta_ksi_est_err_tilt agent 2/4(ksi_est_err_tilt_vec)
  Mux121/1 -> Interpreted MATLAB Function43/1
  cal theta_eta_est_err_tilt agent 3/1(theta_eta_est_err_tilt_1_3) -> [theta_eta_est_err_tilt_1_3]
  Constant279/1 -> Mux129/2
  choose eta_est_err_tilt 6/1(y) -> cal abs 57/1(x)
  [theta_ksi_est_err_tilt_2_vec] -> fixed-time distributed follower desire position observer agent 5/5(theta_ksi_est_err_tilt_2_vec)
  Interpreted MATLAB Function60/1 -> trans to column60/1(x)
  Constant198/1 -> cal theta_eta_est_err_tilt agent 5/1(alfa_theta)
  Constant219/1 -> fixed-time distributed follower desire position observer agent 2/2(l2p)
  Demux68/2 -> Mux91/1
  cal theta_ksi_est_err_tilt agent 4/1(theta_ksi_est_err_tilt_1_4) -> [theta_ksi_est_err_tilt_1_4]
  trans to column56/1(y) -> [eta_est_err_squ_1_node_3], Display90/1
  Constant268/1 -> Mux121/2
  Demux94/2 -> Mux134/1
  [theta_ksi_est_err_tilt_1_vec] -> fixed-time distributed follower desire position observer agent 1/4(theta_ksi_est_err_tilt_1_vec)
  choose eta_est_err_tilt 9/1(y) -> cal abs 60/1(x)
  combine follower desire velocity estimaters/1(eta_d_est_vec) -> [eta_d_est_vec]
  Constant202/1 -> fixed-time distributed follower desire velocity observer agent 2/2(l2v)
  [eta_est_err_squ_1_node_2] -> cal theta_eta_est_err_tilt agent 2/2(eta_est_err_squ_1_node_2)
  Demux96/1 -> Mux87/1
  Constant186/1 -> cal theta_ksi_est_err_tilt agent 5/1(alfa_theta)
  Constant270/1 -> Mux124/2
  Mux119/1 -> ksi_d_est_2/1
  Constant247/1 -> Mux109/2
  trans to column59/1(y) -> [eta_est_err_squ_2_node_5], Display94/1
  Constant214/1 -> Add4/2
  cal abs 46/1(y) -> Mux122/1
  Demux92/1 -> Mux119/1
  Mux87/1 -> ksi_d_est_4/1
  [theta_ksi_est_err_tilt_1_vec] -> fixed-time distributed follower desire position observer agent 5/4(theta_ksi_est_err_tilt_1_vec)
  Constant194/1 -> cal theta_eta_est_err_tilt agent 2/1(alfa_theta)
  Constant273/1 -> Mux123/3
  trans to column46/1(y) -> [ksi_est_err_squ_2_node_3], Display80/1
  [theta_eta_est_err_tilt_2_vec] -> fixed-time distributed follower desire velocity observer agent 3/4(theta_eta_est_err_tilt_2_vec)
  Demux92/2 -> Mux130/1
  [theta_ksi_est_err_tilt_1_4] -> combine lumped follower position observation error/4(theta_ksi_est_err_tilt_1_4)
  Mux94/1 -> eta_d_est_1/3
  [theta_eta_est_err_tilt_1_2] -> combine lumped follower velocity observation error/2(theta_eta_est_err_tilt_1_2)
  Constant208/1 -> Add5/2
  Demux69/1 -> Mux92/1
  [ksi_est_err_tilt_vec] -> choose eta_est_err_tilt 16/1(x)
  Mux122/1 -> Interpreted MATLAB Function44/1
  Mux120/1 -> Interpreted MATLAB Function42/1
  [theta_eta_est_err_tilt_2_vec] -> fixed-time distributed follower desire velocity observer agent 4/4(theta_eta_est_err_tilt_2_vec)
  Mux103/1 -> eta_d_est_4/2
  Constant206/1 -> fixed-time distributed follower desire velocity observer agent 3/1(l1v)
  [ksi_d_est_5] -> combine leader position estimaters/5(ksi_d_est_5)
  cal theta_ksi_est_err_tilt agent 3/1(theta_ksi_est_err_tilt_1_3) -> [theta_ksi_est_err_tilt_1_3]
  [theta_eta_est_err_tilt_1_vec] -> fixed-time distributed follower desire velocity observer agent 3/3(theta_eta_est_err_tilt_1_vec)
  [eta_est_err_tilt_vec] -> choose eta_est_err_tilt 8/1(x)
  [eta_d_est_1] -> combine follower desire velocity estimaters/1(eta_d_est_1)
  Interpreted MATLAB Function54/1 -> trans to column54/1(x)
  Constant207/1 -> Add2/2
  [theta_ksi_est_err_tilt_2_vec] -> fixed-time distributed follower desire position observer agent 1/5(theta_ksi_est_err_tilt_2_vec)
  Demux79/2 -> Mux106/2
  Mux113/1 -> Interpreted MATLAB Function56/1
  Interpreted MATLAB Function45/1 -> trans to column45/1(x)
  Constant272/1 -> Mux123/2
  Constant193/1 -> cal theta_eta_est_err_tilt agent 1/1(alfa_theta)
  cal abs 45/1(y) -> Mux120/1
  [eta_d_est_2] -> combine follower desire velocity estimaters/2(eta_d_est_2)
  fixed-time distributed follower desire velocity observer agent 4/1(d_eta_d_est_4) -> velocity observe Integrator 4/1
  [ksi_d_est_3] -> combine leader position estimaters/3(ksi_d_est_3)
  trans to column41/1(y) -> [eta_est_err_squ_2_node_1], Display76/1
  [ksi0] -> Add9/1
  Demux93/3 -> Mux132/2
  [ksi0] -> Add7/1
  [eta_est_err_squ_2_node_1] -> cal theta_eta_est_err_tilt agent 1/3(eta_est_err_squ_2_node_1)
  [theta_ksi_est_err_tilt_1_vec] -> fixed-time distributed follower desire position observer agent 2/4(theta_ksi_est_err_tilt_1_vec)
  Constant187/1 -> fixed-time distributed follower desire position observer agent 4/1(l1p)
  position observe Integrator 4/1 -> [ksi_d_est_4], Demux96/1
  [eta_est_err_squ_1_node_3] -> cal theta_eta_est_err_tilt agent 3/2(eta_est_err_squ_1_node_3)
  [theta_eta_est_err_tilt_1_1] -> combine lumped follower velocity observation error/1(theta_eta_est_err_tilt_1_1)
  Mux95/1 -> eta_d_est_2/1
  [ksi_est_err_tilt_vec] -> choose eta_est_err_tilt 19/1(x)
  Mux104/1 -> eta_d_est_4/3
  [theta_eta_est_err_tilt_2_2] -> combine lumped follower velocity observation error/7(theta_eta_est_err_tilt_2_2)
  cal abs 57/1(y) -> Mux112/1
  Add8/1 -> Demux97/1
  Interpreted MATLAB Function49/1 -> trans to column49/1(x)
  Constant205/1 -> fixed-time distributed follower desire velocity observer agent 3/2(l2v)
  choose eta_est_err_tilt 14/1(y) -> cal abs 46/1(x)
  Mux100/1 -> eta_d_est_3/2
  Constant261/1 -> Mux114/3
  cal abs 60/1(y) -> Mux118/1
  Constant280/1 -> Mux129/3
  Mux90/1 -> ksi_d_est_5/1
  [eta_est_err_squ_2_node_5] -> cal theta_eta_est_err_tilt agent 5/3(eta_est_err_squ_2_node_5)
  choose eta_est_err_tilt 16/1(y) -> cal abs 48/1(x)
  Demux72/3 -> Mux98/2
  Constant259/1 -> Mux116/3
  Mux127/1 -> Interpreted MATLAB Function49/1
  [eta_est_err_tilt_vec] -> cal theta_eta_est_err_tilt agent 4/4(eta_est_err_tilt_vec)
  [ksi_est_err_squ_1_node_3] -> cal theta_ksi_est_err_tilt agent 3/2(ksi_est_err_squ_1_node_3)
  [theta_eta_est_err_tilt_2_3] -> combine lumped follower velocity observation error/8(theta_eta_est_err_tilt_2_3)
  Interpreted MATLAB Function51/1 -> trans to column51/1(x)
  Constant203/1 -> fixed-time distributed follower desire velocity observer agent 2/1(l1v)
  [theta_ksi_est_err_tilt_2_5] -> combine lumped follower position observation error/10(theta_ksi_est_err_tilt_2_5)
  cal abs 49/1(y) -> Mux123/1
  Constant192/1 -> Add9/2
  [eta_d_est_4] -> combine follower desire velocity estimaters/4(eta_d_est_4)
  [theta_ksi_est_err_tilt_2_vec] -> fixed-time distributed follower desire position observer agent 3/5(theta_ksi_est_err_tilt_2_vec)
  fixed-time distributed follower desire position observer agent 1/1(d_ksi_d_est_1) -> position observe Integrator 1/1
  choose eta_est_err_tilt 18/1(y) -> cal abs 50/1(x)
  Demux76/1 -> Mux102/2
  [eta_est_err_squ_1_node_1] -> cal theta_eta_est_err_tilt agent 1/2(eta_est_err_squ_1_node_1)
  Interpreted MATLAB Function59/1 -> trans to column59/1(x)
  [eta_est_err_tilt_vec] -> choose eta_est_err_tilt 2/1(x)
  choose eta_est_err_tilt 1/1(y) -> cal abs 41/1(x)
  [eta_est_err_tilt_vec] -> choose eta_est_err_tilt 1/1(x)
  trans to column44/1(y) -> [ksi_est_err_squ_1_node_2], Display79/1
  [eta_est_err_tilt_vec] -> cal theta_eta_est_err_tilt agent 3/4(eta_est_err_tilt_vec)
  Demux79/3 -> Mux107/2
  cal theta_ksi_est_err_tilt agent 2/2(theta_ksi_est_err_tilt_2_2) -> [theta_ksi_est_err_tilt_2_2]
  Demux72/2 -> Mux96/2
  [eta0] -> Add/1
  cal abs 48/1(y) -> Mux124/1
  trans to column57/1(y) -> [eta_est_err_squ_2_node_4], Display91/1
  cal theta_eta_est_err_tilt agent 3/2(theta_eta_est_err_tilt_2_3) -> [theta_eta_est_err_tilt_2_3]
  Constant184/1 -> cal theta_ksi_est_err_tilt agent 3/1(alfa_theta)
  Mux98/1 -> eta_d_est_2/3
  Constant220/1 -> Mux122/2
  cal theta_eta_est_err_tilt agent 5/1(theta_eta_est_err_tilt_1_5) -> [theta_eta_est_err_tilt_1_5]
  Demux80/2 -> Mux91/2
  fixed-time distributed follower desire velocity observer agent 2/1(d_eta_d_est_2) -> velocity observe Integrator 2/1
  cal abs 58/1(y) -> Mux116/1
  Demux97/3 -> Mux89/2
  Demux94/3 -> Mux135/1
  Constant266/1 -> Mux117/3
  [eta0] -> cal lumped observation error agent 4/7(eta0)
  cal lumped observation error agent 4/2(eta_est_err_tilt_4) -> [eta_est_err_tilt_4]
  [eta_est_err_tilt_4] -> "combine lumped follower observation error "/9(eta_est_err_tilt_4)
  cal position estimate error/1(ksi_est_err) -> [ksi_est_err]
  cal velocity estimate error/1(eta_est_err) -> [eta_est_err]
  [eta_est_err_tilt_1] -> "combine lumped follower observation error "/6(eta_est_err_tilt_1)
  [eta0] -> cal velocity estimate error/2(eta0)
  [eta_d_est_vec] -> cal velocity estimate error/1(eta_d_est_vec)
  [ksi0] -> cal position estimate error/2(ksi0)
  cal lumped observation error agent 3/2(eta_est_err_tilt_3) -> [eta_est_err_tilt_3]
  Constant242/1 -> cal lumped observation error agent 5/2(w0)
  "combine lumped follower observation error "/2(eta_est_err_tilt_vec) -> [eta_est_err_tilt_vec]
  cal lumped observation error agent 4/1(ksi_est_err_tilt_4) -> [ksi_est_err_tilt_4]
  [ksi_est_err_tilt_3] -> "combine lumped follower observation error "/3(ksi_est_err_tilt_3)
  [delta_eta_vec] -> cal lumped observation error agent 4/8(delta_eta_vec)
  [delta_ksi_vec] -> cal position estimate error/3(delta_ksi_vec)
  Constant240/1 -> cal lumped observation error agent 5/1(wij)
  cal lumped observation error agent 1/1(ksi_est_err_tilt_1) -> [ksi_est_err_tilt_1]
  [delta_eta_vec] -> cal velocity estimate error/3(delta_eta_vec)
  cal lumped observation error agent 2/1(ksi_est_err_tilt_2) -> [ksi_est_err_tilt_2]
  [ksi_d_est_vec] -> cal lumped observation error agent 1/3(ksi_d_est_vec)
  Constant237/1 -> cal lumped observation error agent 4/2(w0)
  [ksi0] -> cal lumped observation error agent 2/4(ksi0)
  [delta_ksi_vec] -> cal lumped observation error agent 5/5(delta_ksi_vec)
  [ksi_est_err_tilt_4] -> "combine lumped follower observation error "/4(ksi_est_err_tilt_4)
  [eta0] -> cal lumped observation error agent 2/7(eta0)
  [delta_eta_vec] -> cal lumped observation error agent 5/8(delta_eta_vec)
  [delta_ksi_vec] -> cal lumped observation error agent 3/5(delta_ksi_vec)
  [delta_eta_vec] -> cal lumped observation error agent 2/8(delta_eta_vec)
  cal lumped observation error agent 1/2(eta_est_err_tilt_1) -> [eta_est_err_tilt_1]
  [eta_d_est_vec] -> cal lumped observation error agent 5/6(eta_d_est_vec)
  [ksi_est_err_tilt_2] -> "combine lumped follower observation error "/2(ksi_est_err_tilt_2)
  [eta_d_est_vec] -> cal lumped observation error agent 3/6(eta_d_est_vec)
  [eta_est_err_tilt_3] -> "combine lumped follower observation error "/8(eta_est_err_tilt_3)
  [delta_ksi_vec] -> cal lumped observation error agent 4/5(delta_ksi_vec)
  Constant224/1 -> cal lumped observation error agent 1/2(w0)
  [delta_ksi_vec] -> cal lumped observation error agent 2/5(delta_ksi_vec)
  [eta_d_est_vec] -> cal lumped observation error agent 2/6(eta_d_est_vec)
  [ksi0] -> cal lumped observation error agent 4/4(ksi0)
  cal lumped observation error agent 5/2(eta_est_err_tilt_5) -> [eta_est_err_tilt_5]
  Constant227/1 -> cal lumped observation error agent 2/1(wij)
  [ksi_d_est_vec] -> cal position estimate error/1(ksi_d_est_vec)
  [ksi_est_err_tilt_5] -> "combine lumped follower observation error "/5(ksi_est_err_tilt_5)
  [ksi0] -> cal lumped observation error agent 3/4(ksi0)
  cal lumped observation error agent 5/1(ksi_est_err_tilt_5) -> [ksi_est_err_tilt_5]
  cal lumped observation error agent 3/1(ksi_est_err_tilt_3) -> [ksi_est_err_tilt_3]
  [delta_eta_vec] -> cal lumped observation error agent 3/8(delta_eta_vec)
  Constant236/1 -> cal lumped observation error agent 4/1(wij)
  Constant232/1 -> cal lumped observation error agent 3/1(wij)
  [ksi0] -> cal lumped observation error agent 5/4(ksi0)
  [eta_est_err_tilt_5] -> "combine lumped follower observation error "/10(eta_est_err_tilt_5)
  [ksi_d_est_vec] -> cal lumped observation error agent 5/3(ksi_d_est_vec)
  "combine lumped follower observation error "/1(ksi_est_err_tilt_vec) -> [ksi_est_err_tilt_vec]
  Constant223/1 -> cal lumped observation error agent 1/1(wij)
  Constant233/1 -> cal lumped observation error agent 3/2(w0)
  [eta0] -> cal lumped observation error agent 1/7(eta0)
  [ksi0] -> cal lumped observation error agent 1/4(ksi0)
  [ksi_d_est_vec] -> cal lumped observation error agent 2/3(ksi_d_est_vec)
  [ksi_d_est_vec] -> cal lumped observation error agent 3/3(ksi_d_est_vec)
  [eta_d_est_vec] -> cal lumped observation error agent 4/6(eta_d_est_vec)
  [ksi_est_err_tilt_1] -> "combine lumped follower observation error "/1(ksi_est_err_tilt_1)
  [delta_ksi_vec] -> cal lumped observation error agent 1/5(delta_ksi_vec)
  cal lumped observation error agent 2/2(eta_est_err_tilt_2) -> [eta_est_err_tilt_2]
  [eta0] -> cal lumped observation error agent 3/7(eta0)
  [delta_eta_vec] -> cal lumped observation error agent 1/8(delta_eta_vec)
  [eta_d_est_vec] -> cal lumped observation error agent 1/6(eta_d_est_vec)
  Constant228/1 -> cal lumped observation error agent 2/2(w0)
  [eta0] -> cal lumped observation error agent 5/7(eta0)
  [ksi_d_est_vec] -> cal lumped observation error agent 4/3(ksi_d_est_vec)
  [eta_est_err_tilt_2] -> "combine lumped follower observation error "/7(eta_est_err_tilt_2)
